simulink model "muv"  (Simulink 8.9)
settings: Solver=VariableStepAuto  StartTime=0.0  StopTime=10.0  RelTol=1e-3
settings Model: Creator=god  LastModifiedBy=muthu
settings DataIOCC: LimitDataPoints=off  SaveFormat=Dataset  SignalLoggingSaveFormat=Dataset
settings OptimizationCC: LifeSpan=auto
settings DebuggingCC: UnderspecifiedInitializationDetection=Simplified  MergeDetectMultiDrivingBlocksExec=error  FcnCallInpInsideContextMsg=error  StateNameClashWarn=none  SFUnexpectedBacktrackingDiag=error  SFNoUnconditionalDefaultTransitionDiag=error  SFExecutionAtInitializationDiag=warning
settings HardwareCC: ProdBitPerPointer=64  ProdBitPerSizeT=64  ProdBitPerPtrDiffT=64  ProdLargestAtomicFloat=Float  ProdIntDivRoundTo=Zero  ProdEndianess=LittleEndian  ProdWordSize=64  ProdHWDeviceType=Intel->x86-64 (Windows64)
settings ModelReferenceCC: PropagateSignalLabelsOutOfModel=on
settings GRTTargetCC: TargetLangStandard=C99 (ISO)  GeneratePreprocessorConditionals=Use local settings  CombineOutputUpdateFcns=on  GRTInterface=off
settings ConfigComp: CovMetricSettings=dwe  CovHtmlReporting=off  CovSaveCumulativeToWorkspaceVar=off  CovSaveSingleToWorkspaceVar=off  CovExternalEMLEnable=on

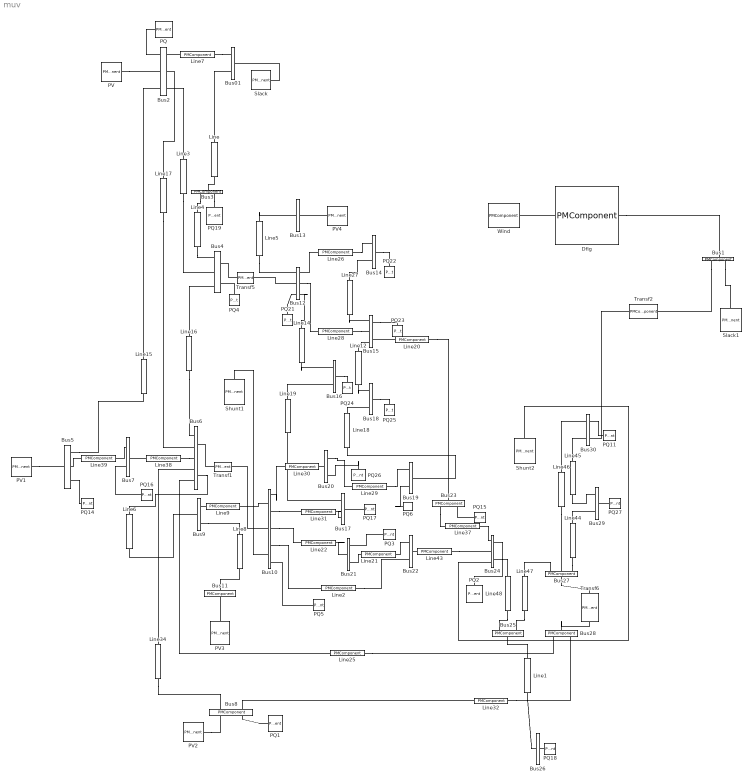
== system muv ==
  Bus01 : PMComponent  Tag=PSATblock  Description=Connection  PhysicalDomain=psatdomain  LeftPortType=p1  RightPortType=p1  LConnTagsString=__newl0  RConnTagsString=__newr0|__newr1  mask(Bus){in=1, out=2, p2q=132, p3_4q=[1.10  0.90], p5q=1, p6q=1}
      mask prompts: in "Number of inputs:"; out "Number of outputs:"; p2q "Voltage Rating [kV]"; p3_4q "Voltage initial guess [p.u.  rad]"; p5q "Area number"; p6q "Region number"
      mask help: Bus block.
      mask init:
      | fm_inout
      mask Callback p5q: fm_block
      mask Display: plot([0 1 1 0 0],[0 0 1 1 0])
  Bus1 : PMComponent  Tag=PSATblock  Description=Connection  PhysicalDomain=psatdomain  LeftPortType=p1  RightPortType=p1  LConnTagsString=__newl0|__newl1  RConnTagsString=__newr0  mask(Bus){in=2, out=1, p2q=33, p3_4q=[1.00  0.00], p5q=1, p6q=1}
      mask prompts: in "Number of inputs:"; out "Number of outputs:"; p2q "Voltage Rating [kV]"; p3_4q "Voltage initial guess [p.u.  rad]"; p5q "Area number"; p6q "Region number"
      mask help: Bus block.
      mask init:
      | fm_inout
      mask Callback p5q: fm_block
      mask Display: plot([0 1 1 0 0],[0 0 1 1 0])
  Bus10 : PMComponent  Tag=PSATblock  Description=Connection  PhysicalDomain=psatdomain  LeftPortType=p1  RightPortType=p1  LConnTagsString=__newl0|__newl1|__newl2  RConnTagsString=__newr0|__newr1|__newr2|__newr3|__newr4  mask(Bus){in=3, out=5, p2q=33, p3_4q=[1.00  0.00], p5q=1, p6q=1}
      mask prompts: in "Number of inputs:"; out "Number of outputs:"; p2q "Voltage Rating [kV]"; p3_4q "Voltage initial guess [p.u.  rad]"; p5q "Area number"; p6q "Region number"
      mask help: Bus block.
      mask init:
      | fm_inout
      mask Callback p5q: fm_block
      mask Display: plot([0 1 1 0 0],[0 0 1 1 0])
  Bus11 : PMComponent  Tag=PSATblock  Description=Connection  PhysicalDomain=psatdomain  LeftPortType=p1  RightPortType=p1  LConnTagsString=__newl0  RConnTagsString=__newr0  mask(Bus){in=1, out=1, p2q=132, p3_4q=[1.00  0.00], p5q=1, p6q=1}
      mask prompts: in "Number of inputs:"; out "Number of outputs:"; p2q "Voltage Rating [kV]"; p3_4q "Voltage initial guess [p.u.  rad]"; p5q "Area number"; p6q "Region number"
      mask help: Bus block.
      mask init:
      | fm_inout
      mask Callback p5q: fm_block
      mask Display: plot([0 1 1 0 0],[0 0 1 1 0])
  Bus12 : PMComponent  Tag=PSATblock  Description=Connection  PhysicalDomain=psatdomain  LeftPortType=p1  RightPortType=p1  LConnTagsString=__newl0|__newl1|__newl2  RConnTagsString=__newr0|__newr1|__newr2  mask(Bus){in=3, out=3, p2q=33, p3_4q=[1.00  0.00], p5q=1, p6q=1}
      mask prompts: in "Number of inputs:"; out "Number of outputs:"; p2q "Voltage Rating [kV]"; p3_4q "Voltage initial guess [p.u.  rad]"; p5q "Area number"; p6q "Region number"
      mask help: Bus block.
      mask init:
      | fm_inout
      mask Callback p5q: fm_block
      mask Display: plot([0 1 1 0 0],[0 0 1 1 0])
  Bus13 : PMComponent  Tag=PSATblock  Description=Connection  PhysicalDomain=psatdomain  LeftPortType=p1  RightPortType=p1  LConnTagsString=__newl0  RConnTagsString=__newr0  mask(Bus){in=1, out=1, p2q=11, p3_4q=[1.00  0.00], p5q=1, p6q=1}
      mask prompts: in "Number of inputs:"; out "Number of outputs:"; p2q "Voltage Rating [kV]"; p3_4q "Voltage initial guess [p.u.  rad]"; p5q "Area number"; p6q "Region number"
      mask help: Bus block.
      mask init:
      | fm_inout
      mask Callback p5q: fm_block
      mask Display: plot([0 1 1 0 0],[0 0 1 1 0])
  Bus14 : PMComponent  Tag=PSATblock  Description=Connection  PhysicalDomain=psatdomain  LeftPortType=p1  RightPortType=p1  LConnTagsString=__newl0|__newl1  RConnTagsString=__newr0  mask(Bus){in=2, out=1, p2q=33, p3_4q=[1.00  0.00], p5q=1, p6q=1}
      mask prompts: in "Number of inputs:"; out "Number of outputs:"; p2q "Voltage Rating [kV]"; p3_4q "Voltage initial guess [p.u.  rad]"; p5q "Area number"; p6q "Region number"
      mask help: Bus block.
      mask init:
      | fm_inout
      mask Callback p5q: fm_block
      mask Display: plot([0 1 1 0 0],[0 0 1 1 0])
  Bus15 : PMComponent  Tag=PSATblock  Description=Connection  PhysicalDomain=psatdomain  LeftPortType=p1  RightPortType=p1  LConnTagsString=__newl0|__newl1|__newl2  RConnTagsString=__newr0|__newr1  mask(Bus){in=3, out=2, p2q=33, p3_4q=[1.00  0.00], p5q=1, p6q=1}
      mask prompts: in "Number of inputs:"; out "Number of outputs:"; p2q "Voltage Rating [kV]"; p3_4q "Voltage initial guess [p.u.  rad]"; p5q "Area number"; p6q "Region number"
      mask help: Bus block.
      mask init:
      | fm_inout
      mask Callback p5q: fm_block
      mask Display: plot([0 1 1 0 0],[0 0 1 1 0])
  Bus16 : PMComponent  Tag=PSATblock  Description=Connection  PhysicalDomain=psatdomain  LeftPortType=p1  RightPortType=p1  LConnTagsString=__newl0|__newl1  RConnTagsString=__newr0  mask(Bus){in=2, out=1, p2q=33, p3_4q=[1.00  0.00], p5q=1, p6q=1}
      mask prompts: in "Number of inputs:"; out "Number of outputs:"; p2q "Voltage Rating [kV]"; p3_4q "Voltage initial guess [p.u.  rad]"; p5q "Area number"; p6q "Region number"
      mask help: Bus block.
      mask init:
      | fm_inout
      mask Callback p5q: fm_block
      mask Display: plot([0 1 1 0 0],[0 0 1 1 0])
  Bus17 : PMComponent  Tag=PSATblock  Description=Connection  PhysicalDomain=psatdomain  LeftPortType=p1  RightPortType=p1  LConnTagsString=__newl0|__newl1  RConnTagsString=__newr0  mask(Bus){in=2, out=1, p2q=33, p3_4q=[1.00  0.00], p5q=1, p6q=1}
      mask prompts: in "Number of inputs:"; out "Number of outputs:"; p2q "Voltage Rating [kV]"; p3_4q "Voltage initial guess [p.u.  rad]"; p5q "Area number"; p6q "Region number"
      mask help: Bus block.
      mask init:
      | fm_inout
      mask Callback p5q: fm_block
      mask Display: plot([0 1 1 0 0],[0 0 1 1 0])
  Bus18 : PMComponent  Tag=PSATblock  Description=Connection  PhysicalDomain=psatdomain  LeftPortType=p1  RightPortType=p1  LConnTagsString=__newl0|__newl1  RConnTagsString=__newr0  mask(Bus){in=2, out=1, p2q=33, p3_4q=[1.00  0.00], p5q=1, p6q=1}
      mask prompts: in "Number of inputs:"; out "Number of outputs:"; p2q "Voltage Rating [kV]"; p3_4q "Voltage initial guess [p.u.  rad]"; p5q "Area number"; p6q "Region number"
      mask help: Bus block.
      mask init:
      | fm_inout
      mask Callback p5q: fm_block
      mask Display: plot([0 1 1 0 0],[0 0 1 1 0])
  Bus19 : PMComponent  Tag=PSATblock  Description=Connection  PhysicalDomain=psatdomain  LeftPortType=p1  RightPortType=p1  LConnTagsString=__newl0|__newl1  RConnTagsString=__newr0  mask(Bus){in=2, out=1, p2q=33, p3_4q=[1.00  0.00], p5q=1, p6q=1}
      mask prompts: in "Number of inputs:"; out "Number of outputs:"; p2q "Voltage Rating [kV]"; p3_4q "Voltage initial guess [p.u.  rad]"; p5q "Area number"; p6q "Region number"
      mask help: Bus block.
      mask init:
      | fm_inout
      mask Callback p5q: fm_block
      mask Display: plot([0 1 1 0 0],[0 0 1 1 0])
  Bus2 : PMComponent  Tag=PSATblock  Description=Connection  PhysicalDomain=psatdomain  LeftPortType=p1  RightPortType=p1  LConnTagsString=__newl0|__newl1|__newl2  RConnTagsString=__newr0|__newr1|__newr2  mask(Bus){in=3, out=3, p2q=132, p3_4q=[1.00  0.00], p5q=1, p6q=1}
      mask prompts: in "Number of inputs:"; out "Number of outputs:"; p2q "Voltage Rating [kV]"; p3_4q "Voltage initial guess [p.u.  rad]"; p5q "Area number"; p6q "Region number"
      mask help: Bus block.
      mask init:
      | fm_inout
      mask Callback p5q: fm_block
      mask Display: plot([0 1 1 0 0],[0 0 1 1 0])
  Bus20 : PMComponent  Tag=PSATblock  Description=Connection  PhysicalDomain=psatdomain  LeftPortType=p1  RightPortType=p1  LConnTagsString=__newl0  RConnTagsString=__newr0|__newr1  mask(Bus){in=1, out=2, p2q=33, p3_4q=[1.00  0.00], p5q=1, p6q=1}
      mask prompts: in "Number of inputs:"; out "Number of outputs:"; p2q "Voltage Rating [kV]"; p3_4q "Voltage initial guess [p.u.  rad]"; p5q "Area number"; p6q "Region number"
      mask help: Bus block.
      mask init:
      | fm_inout
      mask Callback p5q: fm_block
      mask Display: plot([0 1 1 0 0],[0 0 1 1 0])
  Bus21 : PMComponent  Tag=PSATblock  Description=Connection  PhysicalDomain=psatdomain  LeftPortType=p1  RightPortType=p1  LConnTagsString=__newl0  RConnTagsString=__newr0|__newr1  mask(Bus){in=1, out=2, p2q=33, p3_4q=[1.00  0.00], p5q=1, p6q=1}
      mask prompts: in "Number of inputs:"; out "Number of outputs:"; p2q "Voltage Rating [kV]"; p3_4q "Voltage initial guess [p.u.  rad]"; p5q "Area number"; p6q "Region number"
      mask help: Bus block.
      mask init:
      | fm_inout
      mask Callback p5q: fm_block
      mask Display: plot([0 1 1 0 0],[0 0 1 1 0])
  Bus22 : PMComponent  Tag=PSATblock  Description=Connection  PhysicalDomain=psatdomain  LeftPortType=p1  RightPortType=p1  LConnTagsString=__newl0|__newl1  RConnTagsString=__newr0  mask(Bus){in=2, out=1, p2q=33, p3_4q=[1.00  0.00], p5q=1, p6q=1}
      mask prompts: in "Number of inputs:"; out "Number of outputs:"; p2q "Voltage Rating [kV]"; p3_4q "Voltage initial guess [p.u.  rad]"; p5q "Area number"; p6q "Region number"
      mask help: Bus block.
      mask init:
      | fm_inout
      mask Callback p5q: fm_block
      mask Display: plot([0 1 1 0 0],[0 0 1 1 0])
  Bus23 : PMComponent  Tag=PSATblock  Description=Connection  PhysicalDomain=psatdomain  LeftPortType=p1  RightPortType=p1  LConnTagsString=__newl0  RConnTagsString=__newr0|__newr1  mask(Bus){in=1, out=2, p2q=33, p3_4q=[1.00  0.00], p5q=1, p6q=1}
      mask prompts: in "Number of inputs:"; out "Number of outputs:"; p2q "Voltage Rating [kV]"; p3_4q "Voltage initial guess [p.u.  rad]"; p5q "Area number"; p6q "Region number"
      mask help: Bus block.
      mask init:
      | fm_inout
      mask Callback p5q: fm_block
      mask Display: plot([0 1 1 0 0],[0 0 1 1 0])
  Bus24 : PMComponent  Tag=PSATblock  Description=Connection  PhysicalDomain=psatdomain  LeftPortType=p1  RightPortType=p1  LConnTagsString=__newl0|__newl1|__newl2  RConnTagsString=__newr0|__newr1  mask(Bus){in=3, out=2, p2q=32, p3_4q=[1.00  0.00], p5q=1, p6q=1}
      mask prompts: in "Number of inputs:"; out "Number of outputs:"; p2q "Voltage Rating [kV]"; p3_4q "Voltage initial guess [p.u.  rad]"; p5q "Area number"; p6q "Region number"
      mask help: Bus block.
      mask init:
      | fm_inout
      mask Callback p5q: fm_block
      mask Display: plot([0 1 1 0 0],[0 0 1 1 0])
  Bus25 : PMComponent  Tag=PSATblock  Description=Connection  PhysicalDomain=psatdomain  LeftPortType=p1  RightPortType=p1  LConnTagsString=__newl0|__newl1  RConnTagsString=__newr0  mask(Bus){in=2, out=1, p2q=33, p3_4q=[1.00  0.00], p5q=1, p6q=1}
      mask prompts: in "Number of inputs:"; out "Number of outputs:"; p2q "Voltage Rating [kV]"; p3_4q "Voltage initial guess [p.u.  rad]"; p5q "Area number"; p6q "Region number"
      mask help: Bus block.
      mask init:
      | fm_inout
      mask Callback p5q: fm_block
      mask Display: plot([0 1 1 0 0],[0 0 1 1 0])
  Bus26 : PMComponent  Tag=PSATblock  Description=Connection  PhysicalDomain=psatdomain  LeftPortType=p1  RightPortType=p1  LConnTagsString=__newl0  RConnTagsString=__newr0  mask(Bus){in=1, out=1, p2q=33, p3_4q=[1.00  0.00], p5q=1, p6q=1}
      mask prompts: in "Number of inputs:"; out "Number of outputs:"; p2q "Voltage Rating [kV]"; p3_4q "Voltage initial guess [p.u.  rad]"; p5q "Area number"; p6q "Region number"
      mask help: Bus block.
      mask init:
      | fm_inout
      mask Callback p5q: fm_block
      mask Display: plot([0 1 1 0 0],[0 0 1 1 0])
  Bus27 : PMComponent  Tag=PSATblock  Description=Connection  PhysicalDomain=psatdomain  LeftPortType=p1  RightPortType=p1  LConnTagsString=__newl0  RConnTagsString=__newr0|__newr1|__newr2  mask(Bus){in=1, out=3, p2q=33, p3_4q=[1.00  0.00], p5q=1, p6q=1}
      mask prompts: in "Number of inputs:"; out "Number of outputs:"; p2q "Voltage Rating [kV]"; p3_4q "Voltage initial guess [p.u.  rad]"; p5q "Area number"; p6q "Region number"
      mask help: Bus block.
      mask init:
      | fm_inout
      mask Callback p5q: fm_block
      mask Display: plot([0 1 1 0 0],[0 0 1 1 0])
  Bus28 : PMComponent  Tag=PSATblock  Description=Connection  PhysicalDomain=psatdomain  LeftPortType=p1  RightPortType=p1  LConnTagsString=__newl0|__newl1  RConnTagsString=__newr0  mask(Bus){in=2, out=1, p2q=132, p3_4q=[1.00  0.00], p5q=1, p6q=1}
      mask prompts: in "Number of inputs:"; out "Number of outputs:"; p2q "Voltage Rating [kV]"; p3_4q "Voltage initial guess [p.u.  rad]"; p5q "Area number"; p6q "Region number"
      mask help: Bus block.
      mask init:
      | fm_inout
      mask Callback p5q: fm_block
      mask Display: plot([0 1 1 0 0],[0 0 1 1 0])
  Bus29 : PMComponent  Tag=PSATblock  Description=Connection  PhysicalDomain=psatdomain  LeftPortType=p1  RightPortType=p1  LConnTagsString=__newl0|__newl1  RConnTagsString=__newr0  mask(Bus){in=2, out=1, p2q=33, p3_4q=[1.00  0.00], p5q=1, p6q=1}
      mask prompts: in "Number of inputs:"; out "Number of outputs:"; p2q "Voltage Rating [kV]"; p3_4q "Voltage initial guess [p.u.  rad]"; p5q "Area number"; p6q "Region number"
      mask help: Bus block.
      mask init:
      | fm_inout
      mask Callback p5q: fm_block
      mask Display: plot([0 1 1 0 0],[0 0 1 1 0])
  Bus3 : PMComponent  Tag=PSATblock  Description=Connection  PhysicalDomain=psatdomain  LeftPortType=p1  RightPortType=p1  LConnTagsString=__newl0  RConnTagsString=__newr0|__newr1  mask(Bus){in=1, out=2, p2q=132, p3_4q=[1.00  0.00], p5q=1, p6q=1}
      mask prompts: in "Number of inputs:"; out "Number of outputs:"; p2q "Voltage Rating [kV]"; p3_4q "Voltage initial guess [p.u.  rad]"; p5q "Area number"; p6q "Region number"
      mask help: Bus block.
      mask init:
      | fm_inout
      mask Callback p5q: fm_block
      mask Display: plot([0 1 1 0 0],[0 0 1 1 0])
  Bus30 : PMComponent  Tag=PSATblock  Description=Connection  PhysicalDomain=psatdomain  LeftPortType=p1  RightPortType=p1  LConnTagsString=__newl0|__newl1  RConnTagsString=__newr0|__newr1  mask(Bus){in=2, out=2, p2q=33, p3_4q=[1.00  0.00], p5q=1, p6q=1}
      mask prompts: in "Number of inputs:"; out "Number of outputs:"; p2q "Voltage Rating [kV]"; p3_4q "Voltage initial guess [p.u.  rad]"; p5q "Area number"; p6q "Region number"
      mask help: Bus block.
      mask init:
      | fm_inout
      mask Callback p5q: fm_block
      mask Display: plot([0 1 1 0 0],[0 0 1 1 0])
  Bus4 : PMComponent  Tag=PSATblock  Description=Connection  PhysicalDomain=psatdomain  LeftPortType=p1  RightPortType=p1  LConnTagsString=__newl0|__newl1|__newl2  RConnTagsString=__newr0|__newr1  mask(Bus){in=3, out=2, p2q=132, p3_4q=[1   0.00], p5q=1, p6q=1}
      mask prompts: in "Number of inputs:"; out "Number of outputs:"; p2q "Voltage Rating [kV]"; p3_4q "Voltage initial guess [p.u.   rad]"; p5q "Area number"; p6q "Region number"
      mask help: Bus block
      mask init:
      | fm_inout
      mask Callback p5q: fm_block
      mask Display: plot([0 1 1 0 0],[0 0 1 1 0])
  Bus5 : PMComponent  Tag=PSATblock  Description=Connection  PhysicalDomain=psatdomain  LeftPortType=p1  RightPortType=p1  LConnTagsString=__newl0  RConnTagsString=__newr0|__newr1|__newr2  mask(Bus){in=1, out=3, p2q=132, p3_4q=[1.00   0.00], p5q=1, p6q=1}
      mask prompts: in "Number of inputs:"; out "Number of outputs:"; p2q "Voltage Rating [kV]"; p3_4q "Voltage initial guess [p.u.   rad]"; p5q "Area number"; p6q "Region number"
      mask help: Bus block
      mask init:
      | fm_inout
      mask Callback p5q: fm_block
      mask Display: plot([0 1 1 0 0],[0 0 1 1 0])
  Bus6 : PMComponent  Tag=PSATblock  Description=Connection  PhysicalDomain=psatdomain  LeftPortType=p1  RightPortType=p1  LConnTagsString=__newl0|__newl1|__newl2|__newl3|__newl4  RConnTagsString=__newr0|__newr1  mask(Bus){in=5, out=2, p2q=132, p3_4q=[1.00   0.00], p5q=1, p6q=1}
      mask prompts: in "Number of inputs:"; out "Number of outputs:"; p2q "Voltage Rating [kV]"; p3_4q "Voltage initial guess [p.u.   rad]"; p5q "Area number"; p6q "Region number"
      mask help: Bus block
      mask init:
      | fm_inout
      mask Callback p5q: fm_block
      mask Display: plot([0 1 1 0 0],[0 0 1 1 0])
  Bus7 : PMComponent  Tag=PSATblock  Description=Connection  PhysicalDomain=psatdomain  LeftPortType=p1  RightPortType=p1  LConnTagsString=__newl0|__newl1  RConnTagsString=__newr0  mask(Bus){in=2, out=1, p2q=132, p3_4q=[1.00   0.00], p5q=1, p6q=1}
      mask prompts: in "Number of inputs:"; out "Number of outputs:"; p2q "Voltage Rating [kV]"; p3_4q "Voltage initial guess [p.u.   rad]"; p5q "Area number"; p6q "Region number"
      mask help: Bus block
      mask init:
      | fm_inout
      mask Callback p5q: fm_block
      mask Display: plot([0 1 1 0 0],[0 0 1 1 0])
  Bus8 : PMComponent  Tag=PSATblock  Description=Connection  PhysicalDomain=psatdomain  LeftPortType=p1  RightPortType=p1  LConnTagsString=__newl0|__newl1  RConnTagsString=__newr0|__newr1  mask(Bus){in=2, out=2, p2q=132, p3_4q=[1.00   0.00], p5q=1, p6q=1}
      mask prompts: in "Number of inputs:"; out "Number of outputs:"; p2q "Voltage Rating [kV]"; p3_4q "Voltage initial guess [p.u.   rad]"; p5q "Area number"; p6q "Region number"
      mask help: Bus block
      mask init:
      | fm_inout
      mask Callback p5q: fm_block
      mask Display: plot([0 1 1 0 0],[0 0 1 1 0])
  Bus9 : PMComponent  Tag=PSATblock  Description=Connection  PhysicalDomain=psatdomain  LeftPortType=p1  RightPortType=p1  LConnTagsString=__newl0  RConnTagsString=__newr0|__newr1  mask(Bus){in=1, out=2, p2q=1, p3_4q=[1.00  0.00], p5q=1, p6q=1}
      mask prompts: in "Number of inputs:"; out "Number of outputs:"; p2q "Voltage Rating [kV]"; p3_4q "Voltage initial guess [p.u.  rad]"; p5q "Area number"; p6q "Region number"
      mask help: Bus block.
      mask init:
      | fm_inout
      mask Callback p5q: fm_block
      mask Display: plot([0 1 1 0 0],[0 0 1 1 0])
  Dfig : PMComponent  Tag=PSATblock  Description=Wind Turbines  PhysicalDomain=psatdomain  LeftPortType=p1  RightPortType=p1  LConnTagsString=__newl0  RConnTagsString=__newr0  mask(Dfig){p3_4_5q=[100   33   50], p6_7q=[0.01  0.10], p8_9q=[0.01  0.08], p10q=3.00, p11q=3, p12_13q=[10 3], p14q=10, p15q=0.01, p17_19q=[4 1/89], p16_18q=[75.00  3], p20_21q=[1.00  0.00], p22_23q=[0.7  -0.7], p24q=1, p25q=on}
      mask prompts: p3_4_5q "Power, Voltage and Frequency Ratings [MVA, kV, Hz]"; p6_7q "Stator Resistance Rs and Reactance Xs [p.u.  p.u.]"; p8_9q "Rotor Resitance Rr and Reactance Xr [p.u. p.u.]"; p10q "Magnetization Reactance Xm [p.u.]"; p11q "Inertia Constants Hm  [kWs/kVA]"; p12_13q "Pitch control gain and time constant  Kp, Tp [p.u.  s]"; p14q "Voltage control gain Kv [p.u.]"; p15q "Power Control time constant Te [s]"; p17_19q "Number of poles p and gear box ratio [int  -]"; p16_18q "Blade length and number [m int]"; p20_21q "Pmax and Pmin [p.u.  p.u.]"; p22_23q "Qmax and Qmin [p.u.  p.u.]"; p24q "Number of wind generators that compose the park"; p25q "Connected"
      mask help: This block defines a variable speed wind turbine with doubly fed induction generator.
      mask init:
      | [x,y] = fm_draw('circle');
      | [xh,yh] = fm_draw('helix');
      mask Callback p25q: fm_block
      mask Display:
      | plot(1.4*x,1.4*y,[0,-2],[0 0],[-2 -3 -3 -2 -2],[-1 -1 1 1 -1],[-3 -5],[0 0],[1.4 3.5],[0 0],1,4.35,[0 0 1.075],[-1 -3.25 -3.25],[2.05  2.05],[0 -2.15])
      | plot(1.5*[0.3 0.3]+2.5,0.5*[-1.7 2.7]-3.5,1.5*[ -0.95  -0.95]+2.5,0.5*[-1.7 2.7]-3.5,1.5*[0 0.2]+2.5,0.5*[0.5 0.5]-3.5)
      | plot(1.5*[0.3 -0.95]+2.5,0.5*[2.7 2.7]-3.5,1.5*[0.3 -0.95]+2.5,0.5*[-1.7 -1.7]-3.5)
      | color('blue')
      | plot(x,y)
      | color('cyan')
      | plot(xh-4,3*yh)
      | color('magenta')
      | plot(1.5*[0 0]+2.5,0.5*[-0.5 1.5]-3.5,1.5*[0 -0.2]+2.5,0.5*[-0.5 -0.5]-3.5,1.5*[0 -0.65]+2.5,0.5*[1.5 1.5]-3.5)
      | plot(1.5*[-0.2 -0.2]+2.5,0.5*[-1 0]-3.5,1.5*[-0.2 -0.45]+2.5,0.5*[-1 -0.5]-3.5,1.5*[-0.2 -0.45]+2.5,0.5*[0 -0.5]-3.5,1.5*[-0.45 -0.45]+2.5,0.5*[-1 0]-3.5)
      | plot(1.5*[-0.2 -0.2]+2.5,0.5*[2 1]-3.5,1.5*[-0.45 -0.45]+2.5,0.5*[2 1]-3.5,1.5*[-0.45 -0.2]+2.5,0.5*[2 1.5]-3.5,1.5*[-0.45 -0.2]+2.5,0.5*[1 1.5]-3.5)
      | plot(1.5*[-0.65 -0.65]+2.5,0.5*[-0.5 1.5]-3.5,1.5*[-0.45 -0.65]+2.5,0.5*[-0.5 -0.5]-3.5,1.5*[-0.45 -0.65]+2.5,0.5*[1.5 1.5]-3.5)
      | plot(1.5*[-0.65 -0.85]+2.5,0.5*[0.5 0.5]-3.5,1.5*[-0.3 -0.3]+2.5,0.5*[1.7 2.2]-3.5,1.5*[-0.325 -0.275]+2.5,0.5*[1.975 1.975]-3.5)
  Line : PMComponent  Tag=PSATblock  Description=Power Flow  PhysicalDomain=psatdomain  LeftPortType=p1  RightPortType=p1  LConnTagsString=__newl0  RConnTagsString=__newr0  mask(Line){p3_4_5q=[130  132 50], p6q=0, p8q=0.0452, p9q=0.1852, p10q=0.04080, p13_14_15q=[0.0  0.0  0.0], p16q=on}
      mask prompts: p3_4_5q "Power, Voltage and Frequency Ratings [MVA, kV, Hz]"; p6q "Length of line [km] (0 for p.u. parameters)"; p8q "Resistance [p.u. (Ohms/km)]"; p9q "Reactance [p.u. (H/km)]"; p10q "Susceptance [p.u. (F/km)]"; p13_14_15q "Imax, Pmax and Smax [p.u., p.u., p.u.]"; p16q "Connected"
      mask help: This block defines a pi model for a tree phase line.
      mask init:
      | [xp,yp] = fm_draw('pi');
      mask Callback p16q: fm_block
      mask Display:
      | plot([-1  1  1 -1 -1],[-0.2 -0.2 0.2 0.2 -0.2])
      | color('blue')
      | plot(0.35*xp,0.2*yp)
  Line1 : PMComponent  Tag=PSATblock  Description=Power Flow  PhysicalDomain=psatdomain  LeftPortType=p1  RightPortType=p1  LConnTagsString=__newl0  RConnTagsString=__newr0  mask(Line){p3_4_5q=[16 33 50], p6q=0, p8q=0.05, p9q=0.10, p10q=0, p13_14_15q=[0.0  0.0  0.0], p16q=on}
      mask prompts: p3_4_5q "Power, Voltage and Frequency Ratings [MVA, kV, Hz]"; p6q "Length of line [km] (0 for p.u. parameters)"; p8q "Resistance [p.u. (Ohms/km)]"; p9q "Reactance [p.u. (H/km)]"; p10q "Susceptance [p.u. (F/km)]"; p13_14_15q "Imax, Pmax and Smax [p.u., p.u., p.u.]"; p16q "Connected"
      mask help: This block defines a pi model for a tree phase line.
      mask init:
      | [xp,yp] = fm_draw('pi');
      mask Callback p16q: fm_block
      mask Display:
      | plot([-1  1  1 -1 -1],[-0.2 -0.2 0.2 0.2 -0.2])
      | color('blue')
      | plot(0.35*xp,0.2*yp)
  Line12 : PMComponent  Tag=PSATblock  Description=Power Flow  PhysicalDomain=psatdomain  LeftPortType=p1  RightPortType=p1  LConnTagsString=__newl0  RConnTagsString=__newr0  mask(Line){p3_4_5q=[16 33  50], p6q=0, p8q=0.1073, p9q=0.2185, p10q=0, p13_14_15q=[0.0  0.0  0.0], p16q=on}
      mask prompts: p3_4_5q "Power, Voltage and Frequency Ratings [MVA, kV, Hz]"; p6q "Length of line [km] (0 for p.u. parameters)"; p8q "Resistance [p.u. (Ohms/km)]"; p9q "Reactance [p.u. (H/km)]"; p10q "Susceptance [p.u. (F/km)]"; p13_14_15q "Imax, Pmax and Smax [p.u., p.u., p.u.]"; p16q "Connected"
      mask help: This block defines a pi model for a tree phase line.
      mask init:
      | [xp,yp] = fm_draw('pi');
      mask Callback p16q: fm_block
      mask Display:
      | plot([-1  1  1 -1 -1],[-0.2 -0.2 0.2 0.2 -0.2])
      | color('blue')
      | plot(0.35*xp,0.2*yp)
  Line14 : PMComponent  Tag=PSATblock  Description=Power Flow  PhysicalDomain=psatdomain  LeftPortType=p1  RightPortType=p1  LConnTagsString=__newl0  RConnTagsString=__newr0  mask(Line){p3_4_5q=[32  33  50], p6q=0, p8q=0.0945, p9q=0.1987, p10q=0, p13_14_15q=[0.0  0.0  0.0], p16q=on}
      mask prompts: p3_4_5q "Power, Voltage and Frequency Ratings [MVA, kV, Hz]"; p6q "Length of line [km] (0 for p.u. parameters)"; p8q "Resistance [p.u. (Ohms/km)]"; p9q "Reactance [p.u. (H/km)]"; p10q "Susceptance [p.u. (F/km)]"; p13_14_15q "Imax, Pmax and Smax [p.u., p.u., p.u.]"; p16q "Connected"
      mask help: This block defines a pi model for a tree phase line.
      mask init:
      | [xp,yp] = fm_draw('pi');
      mask Callback p16q: fm_block
      mask Display:
      | plot([-1  1  1 -1 -1],[-0.2 -0.2 0.2 0.2 -0.2])
      | color('blue')
      | plot(0.35*xp,0.2*yp)
  Line15 : PMComponent  Tag=PSATblock  Description=Power Flow  PhysicalDomain=psatdomain  LeftPortType=p1  RightPortType=p1  LConnTagsString=__newl0  RConnTagsString=__newr0  mask(Line){p3_4_5q=[130 132 50], p6q=0, p8q=0.0472, p9q=0.1983, p10q=0.0418, p13_14_15q=[0.0  0.0  0.0], p16q=on}
      mask prompts: p3_4_5q "Power, Voltage and Frequency Ratings [MVA, kV, Hz]"; p6q "Length of line [km] (0 for p.u. parameters)"; p8q "Resistance [p.u. (Ohms/km)]"; p9q "Reactance [p.u. (H/km)]"; p10q "Susceptance [p.u. (F/km)]"; p13_14_15q "Imax, Pmax and Smax [p.u., p.u., p.u.]"; p16q "Connected"
      mask help: This block defines a pi model for a tree phase line.
      mask init:
      | [xp,yp] = fm_draw('pi');
      mask Callback p16q: fm_block
      mask Display:
      | plot([-1  1  1 -1 -1],[-0.2 -0.2 0.2 0.2 -0.2])
      | color('blue')
      | plot(0.35*xp,0.2*yp)
  Line16 : PMComponent  Tag=PSATblock  Description=Power Flow  PhysicalDomain=psatdomain  LeftPortType=p1  RightPortType=p1  LConnTagsString=__newl0  RConnTagsString=__newr0  mask(Line){p3_4_5q=[90  132  50], p6q=0, p8q=0.0119, p9q=0.0414, p10q=0.0045, p13_14_15q=[0.0  0.0  0.0], p16q=on}
      mask prompts: p3_4_5q "Power, Voltage and Frequency Ratings [MVA, kV, Hz]"; p6q "Length of line [km] (0 for p.u. parameters)"; p8q "Resistance [p.u. (Ohms/km)]"; p9q "Reactance [p.u. (H/km)]"; p10q "Susceptance [p.u. (F/km)]"; p13_14_15q "Imax, Pmax and Smax [p.u., p.u., p.u.]"; p16q "Connected"
      mask help: This block defines a pi model for a tree phase line.
      mask init:
      | [xp,yp] = fm_draw('pi');
      mask Callback p16q: fm_block
      mask Display:
      | plot([-1  1  1 -1 -1],[-0.2 -0.2 0.2 0.2 -0.2])
      | color('blue')
      | plot(0.35*xp,0.2*yp)
  Line17 : PMComponent  Tag=PSATblock  Description=Power Flow  PhysicalDomain=psatdomain  LeftPortType=p1  RightPortType=p1  LConnTagsString=__newl0  RConnTagsString=__newr0  mask(Line){p3_4_5q=[65  132  50], p6q=0, p8q=0.0581, p9q=0.1763, p10q=0.0374, p13_14_15q=[0.0  0.0  0.0], p16q=on}
      mask prompts: p3_4_5q "Power, Voltage and Frequency Ratings [MVA, kV, Hz]"; p6q "Length of line [km] (0 for p.u. parameters)"; p8q "Resistance [p.u. (Ohms/km)]"; p9q "Reactance [p.u. (H/km)]"; p10q "Susceptance [p.u. (F/km)]"; p13_14_15q "Imax, Pmax and Smax [p.u., p.u., p.u.]"; p16q "Connected"
      mask help: This block defines a pi model for a tree phase line.
      mask init:
      | [xp,yp] = fm_draw('pi');
      mask Callback p16q: fm_block
      mask Display:
      | plot([-1  1  1 -1 -1],[-0.2 -0.2 0.2 0.2 -0.2])
      | color('blue')
      | plot(0.35*xp,0.2*yp)
  Line18 : PMComponent  Tag=PSATblock  Description=Power Flow  PhysicalDomain=psatdomain  LeftPortType=p1  RightPortType=p1  LConnTagsString=__newl0  RConnTagsString=__newr0  mask(Line){p3_4_5q=[16 33  50], p6q=0, p8q=0.0639, p9q=0.1292, p10q=0, p13_14_15q=[0.0  0.0  0.0], p16q=on}
      mask prompts: p3_4_5q "Power, Voltage and Frequency Ratings [MVA, kV, Hz]"; p6q "Length of line [km] (0 for p.u. parameters)"; p8q "Resistance [p.u. (Ohms/km)]"; p9q "Reactance [p.u. (H/km)]"; p10q "Susceptance [p.u. (F/km)]"; p13_14_15q "Imax, Pmax and Smax [p.u., p.u., p.u.]"; p16q "Connected"
      mask help: This block defines a pi model for a tree phase line.
      mask init:
      | [xp,yp] = fm_draw('pi');
      mask Callback p16q: fm_block
      mask Display:
      | plot([-1  1  1 -1 -1],[-0.2 -0.2 0.2 0.2 -0.2])
      | color('blue')
      | plot(0.35*xp,0.2*yp)
  Line19 : PMComponent  Tag=PSATblock  Description=Power Flow  PhysicalDomain=psatdomain  LeftPortType=p1  RightPortType=p1  LConnTagsString=__newl0  RConnTagsString=__newr0  mask(Line){p3_4_5q=[16  33  50], p6q=0, p8q=0.0824, p9q=0.1932, p10q=0, p13_14_15q=[0.0  0.0  0.0], p16q=on}
      mask prompts: p3_4_5q "Power, Voltage and Frequency Ratings [MVA, kV, Hz]"; p6q "Length of line [km] (0 for p.u. parameters)"; p8q "Resistance [p.u. (Ohms/km)]"; p9q "Reactance [p.u. (H/km)]"; p10q "Susceptance [p.u. (F/km)]"; p13_14_15q "Imax, Pmax and Smax [p.u., p.u., p.u.]"; p16q "Connected"
      mask help: This block defines a pi model for a tree phase line.
      mask init:
      | [xp,yp] = fm_draw('pi');
      mask Callback p16q: fm_block
      mask Display:
      | plot([-1  1  1 -1 -1],[-0.2 -0.2 0.2 0.2 -0.2])
      | color('blue')
      | plot(0.35*xp,0.2*yp)
  Line2 : PMComponent  Tag=PSATblock  Description=Power Flow  PhysicalDomain=psatdomain  LeftPortType=p1  RightPortType=p1  LConnTagsString=__newl0  RConnTagsString=__newr0  mask(Line){p3_4_5q=[32 33  50], p6q=0, p8q=0.0727, p9q=0.1499, p10q=0, p13_14_15q=[0.0  0.0  0.0], p16q=on}
      mask prompts: p3_4_5q "Power, Voltage and Frequency Ratings [MVA, kV, Hz]"; p6q "Length of line [km] (0 for p.u. parameters)"; p8q "Resistance [p.u. (Ohms/km)]"; p9q "Reactance [p.u. (H/km)]"; p10q "Susceptance [p.u. (F/km)]"; p13_14_15q "Imax, Pmax and Smax [p.u., p.u., p.u.]"; p16q "Connected"
      mask help: This block defines a pi model for a tree phase line.
      mask init:
      | [xp,yp] = fm_draw('pi');
      mask Callback p16q: fm_block
      mask Display:
      | plot([-1  1  1 -1 -1],[-0.2 -0.2 0.2 0.2 -0.2])
      | color('blue')
      | plot(0.35*xp,0.2*yp)
  Line20 : PMComponent  Tag=PSATblock  Description=Power Flow  PhysicalDomain=psatdomain  LeftPortType=p1  RightPortType=p1  LConnTagsString=__newl0  RConnTagsString=__newr0  mask(Line){p3_4_5q=[16  33  50], p6q=0, p8q=0, p9q=0.202, p10q=0, p13_14_15q=[0.0  0.0  0.0], p16q=on}
      mask prompts: p3_4_5q "Power, Voltage and Frequency Ratings [MVA, kV, Hz]"; p6q "Length of line [km] (0 for p.u. parameters)"; p8q "Resistance [p.u. (Ohms/km)]"; p9q "Reactance [p.u. (H/km)]"; p10q "Susceptance [p.u. (F/km)]"; p13_14_15q "Imax, Pmax and Smax [p.u., p.u., p.u.]"; p16q "Connected"
      mask help: This block defines a pi model for a tree phase line.
      mask init:
      | [xp,yp] = fm_draw('pi');
      mask Callback p16q: fm_block
      mask Display:
      | plot([-1  1  1 -1 -1],[-0.2 -0.2 0.2 0.2 -0.2])
      | color('blue')
      | plot(0.35*xp,0.2*yp)
  Line21 : PMComponent  Tag=PSATblock  Description=Power Flow  PhysicalDomain=psatdomain  LeftPortType=p1  RightPortType=p1  LConnTagsString=__newl0  RConnTagsString=__newr0  mask(Line){p3_4_5q=[32 33  50], p6q=0, p8q=0.0116, p9q=0.0236, p10q=0, p13_14_15q=[0.0  0.0  0.0], p16q=on}
      mask prompts: p3_4_5q "Power, Voltage and Frequency Ratings [MVA, kV, Hz]"; p6q "Length of line [km] (0 for p.u. parameters)"; p8q "Resistance [p.u. (Ohms/km)]"; p9q "Reactance [p.u. (H/km)]"; p10q "Susceptance [p.u. (F/km)]"; p13_14_15q "Imax, Pmax and Smax [p.u., p.u., p.u.]"; p16q "Connected"
      mask help: This block defines a pi model for a tree phase line.
      mask init:
      | [xp,yp] = fm_draw('pi');
      mask Callback p16q: fm_block
      mask Display:
      | plot([-1  1  1 -1 -1],[-0.2 -0.2 0.2 0.2 -0.2])
      | color('blue')
      | plot(0.35*xp,0.2*yp)
  Line22 : PMComponent  Tag=PSATblock  Description=Power Flow  PhysicalDomain=psatdomain  LeftPortType=p1  RightPortType=p1  LConnTagsString=__newl0  RConnTagsString=__newr0  mask(Line){p3_4_5q=[32  33  50], p6q=0, p8q=0.0348, p9q=0.0749, p10q=0, p13_14_15q=[0.0  0.0  0.0], p16q=on}
      mask prompts: p3_4_5q "Power, Voltage and Frequency Ratings [MVA, kV, Hz]"; p6q "Length of line [km] (0 for p.u. parameters)"; p8q "Resistance [p.u. (Ohms/km)]"; p9q "Reactance [p.u. (H/km)]"; p10q "Susceptance [p.u. (F/km)]"; p13_14_15q "Imax, Pmax and Smax [p.u., p.u., p.u.]"; p16q "Connected"
      mask help: This block defines a pi model for a tree phase line.
      mask init:
      | [xp,yp] = fm_draw('pi');
      mask Callback p16q: fm_block
      mask Display:
      | plot([-1  1  1 -1 -1],[-0.2 -0.2 0.2 0.2 -0.2])
      | color('blue')
      | plot(0.35*xp,0.2*yp)
  Line25 : PMComponent  Tag=PSATblock  Description=Power Flow  PhysicalDomain=psatdomain  LeftPortType=p1  RightPortType=p1  LConnTagsString=__newl0  RConnTagsString=__newr0  mask(Line){p3_4_5q=[32 132 50], p6q=0, p8q=0.0169, p9q=0.0599, p10q=0.013, p13_14_15q=[0.0  0.0  0.0], p16q=on}
      mask prompts: p3_4_5q "Power, Voltage and Frequency Ratings [MVA, kV, Hz]"; p6q "Length of line [km] (0 for p.u. parameters)"; p8q "Resistance [p.u. (Ohms/km)]"; p9q "Reactance [p.u. (H/km)]"; p10q "Susceptance [p.u. (F/km)]"; p13_14_15q "Imax, Pmax and Smax [p.u., p.u., p.u.]"; p16q "Connected"
      mask help: This block defines a pi model for a tree phase line.
      mask init:
      | [xp,yp] = fm_draw('pi');
      mask Callback p16q: fm_block
      mask Display:
      | plot([-1  1  1 -1 -1],[-0.2 -0.2 0.2 0.2 -0.2])
      | color('blue')
      | plot(0.35*xp,0.2*yp)
  Line26 : PMComponent  Tag=PSATblock  Description=Power Flow  PhysicalDomain=psatdomain  LeftPortType=p1  RightPortType=p1  LConnTagsString=__newl0  RConnTagsString=__newr0  mask(Line){p3_4_5q=[32  33 50], p6q=0, p8q=0.1231, p9q=0.2559, p10q=0, p13_14_15q=[0.0  0.0  0.0], p16q=on}
      mask prompts: p3_4_5q "Power, Voltage and Frequency Ratings [MVA, kV, Hz]"; p6q "Length of line [km] (0 for p.u. parameters)"; p8q "Resistance [p.u. (Ohms/km)]"; p9q "Reactance [p.u. (H/km)]"; p10q "Susceptance [p.u. (F/km)]"; p13_14_15q "Imax, Pmax and Smax [p.u., p.u., p.u.]"; p16q "Connected"
      mask help: This block defines a pi model for a tree phase line.
      mask init:
      | [xp,yp] = fm_draw('pi');
      mask Callback p16q: fm_block
      mask Display:
      | plot([-1  1  1 -1 -1],[-0.2 -0.2 0.2 0.2 -0.2])
      | color('blue')
      | plot(0.35*xp,0.2*yp)
  Line27 : PMComponent  Tag=PSATblock  Description=Power Flow  PhysicalDomain=psatdomain  LeftPortType=p1  RightPortType=p1  LConnTagsString=__newl0  RConnTagsString=__newr0  mask(Line){p3_4_5q=[16  33  50], p6q=0, p8q=0.221, p9q=0.1997, p10q=0, p13_14_15q=[0.0  0.0  0.0], p16q=on}
      mask prompts: p3_4_5q "Power, Voltage and Frequency Ratings [MVA, kV, Hz]"; p6q "Length of line [km] (0 for p.u. parameters)"; p8q "Resistance [p.u. (Ohms/km)]"; p9q "Reactance [p.u. (H/km)]"; p10q "Susceptance [p.u. (F/km)]"; p13_14_15q "Imax, Pmax and Smax [p.u., p.u., p.u.]"; p16q "Connected"
      mask help: This block defines a pi model for a tree phase line.
      mask init:
      | [xp,yp] = fm_draw('pi');
      mask Callback p16q: fm_block
      mask Display:
      | plot([-1  1  1 -1 -1],[-0.2 -0.2 0.2 0.2 -0.2])
      | color('blue')
      | plot(0.35*xp,0.2*yp)
  Line28 : PMComponent  Tag=PSATblock  Description=Power Flow  PhysicalDomain=psatdomain  LeftPortType=p1  RightPortType=p1  LConnTagsString=__newl0  RConnTagsString=__newr0  mask(Line){p3_4_5q=[32  33  50], p6q=0, p8q=0.0662, p9q=0.1304, p10q=0, p13_14_15q=[0.0  0.0  0.0], p16q=on}
      mask prompts: p3_4_5q "Power, Voltage and Frequency Ratings [MVA, kV, Hz]"; p6q "Length of line [km] (0 for p.u. parameters)"; p8q "Resistance [p.u. (Ohms/km)]"; p9q "Reactance [p.u. (H/km)]"; p10q "Susceptance [p.u. (F/km)]"; p13_14_15q "Imax, Pmax and Smax [p.u., p.u., p.u.]"; p16q "Connected"
      mask help: This block defines a pi model for a tree phase line.
      mask init:
      | [xp,yp] = fm_draw('pi');
      mask Callback p16q: fm_block
      mask Display:
      | plot([-1  1  1 -1 -1],[-0.2 -0.2 0.2 0.2 -0.2])
      | color('blue')
      | plot(0.35*xp,0.2*yp)
  Line29 : PMComponent  Tag=PSATblock  Description=Power Flow  PhysicalDomain=psatdomain  LeftPortType=p1  RightPortType=p1  LConnTagsString=__newl0  RConnTagsString=__newr0  mask(Line){p3_4_5q=[32  33  50], p6q=0, p8q=0.034, p9q=0.068, p10q=0, p13_14_15q=[0.0  0.0  0.0], p16q=on}
      mask prompts: p3_4_5q "Power, Voltage and Frequency Ratings [MVA, kV, Hz]"; p6q "Length of line [km] (0 for p.u. parameters)"; p8q "Resistance [p.u. (Ohms/km)]"; p9q "Reactance [p.u. (H/km)]"; p10q "Susceptance [p.u. (F/km)]"; p13_14_15q "Imax, Pmax and Smax [p.u., p.u., p.u.]"; p16q "Connected"
      mask help: This block defines a pi model for a tree phase line.
      mask init:
      | [xp,yp] = fm_draw('pi');
      mask Callback p16q: fm_block
      mask Display:
      | plot([-1  1  1 -1 -1],[-0.2 -0.2 0.2 0.2 -0.2])
      | color('blue')
      | plot(0.35*xp,0.2*yp)
  Line3 : PMComponent  Tag=PSATblock  Description=Power Flow  PhysicalDomain=psatdomain  LeftPortType=p1  RightPortType=p1  LConnTagsString=__newl0  RConnTagsString=__newr0  mask(Line){p3_4_5q=[65  130  50], p6q=0, p8q=0.057, p9q=0.1737, p10q=0.0368, p13_14_15q=[0.0  0.0  0.0], p16q=on}
      mask prompts: p3_4_5q "Power, Voltage and Frequency Ratings [MVA, kV, Hz]"; p6q "Length of line [km] (0 for p.u. parameters)"; p8q "Resistance [p.u. (Ohms/km)]"; p9q "Reactance [p.u. (H/km)]"; p10q "Susceptance [p.u. (F/km)]"; p13_14_15q "Imax, Pmax and Smax [p.u., p.u., p.u.]"; p16q "Connected"
      mask help: This block defines a pi model for a tree phase line.
      mask init:
      | [xp,yp] = fm_draw('pi');
      mask Callback p16q: fm_block
      mask Display:
      | plot([-1  1  1 -1 -1],[-0.2 -0.2 0.2 0.2 -0.2])
      | color('blue')
      | plot(0.35*xp,0.2*yp)
  Line30 : PMComponent  Tag=PSATblock  Description=Power Flow  PhysicalDomain=psatdomain  LeftPortType=p1  RightPortType=p1  LConnTagsString=__newl0  RConnTagsString=__newr0  mask(Line){p3_4_5q=[32  33  50], p6q=0, p8q=0.0936, p9q=0.209, p10q=0, p13_14_15q=[0.0  0.0  0.0], p16q=on}
      mask prompts: p3_4_5q "Power, Voltage and Frequency Ratings [MVA, kV, Hz]"; p6q "Length of line [km] (0 for p.u. parameters)"; p8q "Resistance [p.u. (Ohms/km)]"; p9q "Reactance [p.u. (H/km)]"; p10q "Susceptance [p.u. (F/km)]"; p13_14_15q "Imax, Pmax and Smax [p.u., p.u., p.u.]"; p16q "Connected"
      mask help: This block defines a pi model for a tree phase line.
      mask init:
      | [xp,yp] = fm_draw('pi');
      mask Callback p16q: fm_block
      mask Display:
      | plot([-1  1  1 -1 -1],[-0.2 -0.2 0.2 0.2 -0.2])
      | color('blue')
      | plot(0.35*xp,0.2*yp)
  Line31 : PMComponent  Tag=PSATblock  Description=Power Flow  PhysicalDomain=psatdomain  LeftPortType=p1  RightPortType=p1  LConnTagsString=__newl0  RConnTagsString=__newr0  mask(Line){p3_4_5q=[32  33  50], p6q=0, p8q=0.0324, p9q=0.0845, p10q=0, p13_14_15q=[0.0  0.0  0.0], p16q=on}
      mask prompts: p3_4_5q "Power, Voltage and Frequency Ratings [MVA, kV, Hz]"; p6q "Length of line [km] (0 for p.u. parameters)"; p8q "Resistance [p.u. (Ohms/km)]"; p9q "Reactance [p.u. (H/km)]"; p10q "Susceptance [p.u. (F/km)]"; p13_14_15q "Imax, Pmax and Smax [p.u., p.u., p.u.]"; p16q "Connected"
      mask help: This block defines a pi model for a tree phase line.
      mask init:
      | [xp,yp] = fm_draw('pi');
      mask Callback p16q: fm_block
      mask Display:
      | plot([-1  1  1 -1 -1],[-0.2 -0.2 0.2 0.2 -0.2])
      | color('blue')
      | plot(0.35*xp,0.2*yp)
  Line32 : PMComponent  Tag=PSATblock  Description=Power Flow  PhysicalDomain=psatdomain  LeftPortType=p1  RightPortType=p1  LConnTagsString=__newl0  RConnTagsString=__newr0  mask(Line){p3_4_5q=[32 132 50], p6q=0, p8q=0.0636, p9q=0.2, p10q=0.0428, p13_14_15q=[0.0  0.0  0.0], p16q=on}
      mask prompts: p3_4_5q "Power, Voltage and Frequency Ratings [MVA, kV, Hz]"; p6q "Length of line [km] (0 for p.u. parameters)"; p8q "Resistance [p.u. (Ohms/km)]"; p9q "Reactance [p.u. (H/km)]"; p10q "Susceptance [p.u. (F/km)]"; p13_14_15q "Imax, Pmax and Smax [p.u., p.u., p.u.]"; p16q "Connected"
      mask help: This block defines a pi model for a tree phase line.
      mask init:
      | [xp,yp] = fm_draw('pi');
      mask Callback p16q: fm_block
      mask Display:
      | plot([-1  1  1 -1 -1],[-0.2 -0.2 0.2 0.2 -0.2])
      | color('blue')
      | plot(0.35*xp,0.2*yp)
  Line34 : PMComponent  Tag=PSATblock  Description=Power Flow  PhysicalDomain=psatdomain  LeftPortType=p1  RightPortType=p1  LConnTagsString=__newl0  RConnTagsString=__newr0  mask(Line){p3_4_5q=[32  132  50], p6q=0, p8q=0.012, p9q=0.042, p10q=0.009, p13_14_15q=[0.0  0.0  0.0], p16q=on}
      mask prompts: p3_4_5q "Power, Voltage and Frequency Ratings [MVA, kV, Hz]"; p6q "Length of line [km] (0 for p.u. parameters)"; p8q "Resistance [p.u. (Ohms/km)]"; p9q "Reactance [p.u. (H/km)]"; p10q "Susceptance [p.u. (F/km)]"; p13_14_15q "Imax, Pmax and Smax [p.u., p.u., p.u.]"; p16q "Connected"
      mask help: This block defines a pi model for a tree phase line.
      mask init:
      | [xp,yp] = fm_draw('pi');
      mask Callback p16q: fm_block
      mask Display:
      | plot([-1  1  1 -1 -1],[-0.2 -0.2 0.2 0.2 -0.2])
      | color('blue')
      | plot(0.35*xp,0.2*yp)
  Line37 : PMComponent  Tag=PSATblock  Description=Power Flow  PhysicalDomain=psatdomain  LeftPortType=p1  RightPortType=p1  LConnTagsString=__newl0  RConnTagsString=__newr0  mask(Line){p3_4_5q=[16 33  50], p6q=0, p8q=0.12, p9q=0, p10q=0, p13_14_15q=[0.0  0.0  0.0], p16q=on}
      mask prompts: p3_4_5q "Power, Voltage and Frequency Ratings [MVA, kV, Hz]"; p6q "Length of line [km] (0 for p.u. parameters)"; p8q "Resistance [p.u. (Ohms/km)]"; p9q "Reactance [p.u. (H/km)]"; p10q "Susceptance [p.u. (F/km)]"; p13_14_15q "Imax, Pmax and Smax [p.u., p.u., p.u.]"; p16q "Connected"
      mask help: This block defines a pi model for a tree phase line.
      mask init:
      | [xp,yp] = fm_draw('pi');
      mask Callback p16q: fm_block
      mask Display:
      | plot([-1  1  1 -1 -1],[-0.2 -0.2 0.2 0.2 -0.2])
      | color('blue')
      | plot(0.35*xp,0.2*yp)
  Line38 : PMComponent  Tag=PSATblock  Description=Power Flow  PhysicalDomain=psatdomain  LeftPortType=p1  RightPortType=p1  LConnTagsString=__newl0  RConnTagsString=__newr0  mask(Line){p3_4_5q=[130  132  50], p6q=0, p8q=0.0267, p9q=0.082, p10q=0.017, p13_14_15q=[0.0  0.0  0.0], p16q=on}
      mask prompts: p3_4_5q "Power, Voltage and Frequency Ratings [MVA, kV, Hz]"; p6q "Length of line [km] (0 for p.u. parameters)"; p8q "Resistance [p.u. (Ohms/km)]"; p9q "Reactance [p.u. (H/km)]"; p10q "Susceptance [p.u. (F/km)]"; p13_14_15q "Imax, Pmax and Smax [p.u., p.u., p.u.]"; p16q "Connected"
      mask help: This block defines a pi model for a tree phase line.
      mask init:
      | [xp,yp] = fm_draw('pi');
      mask Callback p16q: fm_block
      mask Display:
      | plot([-1  1  1 -1 -1],[-0.2 -0.2 0.2 0.2 -0.2])
      | color('blue')
      | plot(0.35*xp,0.2*yp)
  Line39 : PMComponent  Tag=PSATblock  Description=Power Flow  PhysicalDomain=psatdomain  LeftPortType=p1  RightPortType=p1  LConnTagsString=__newl0  RConnTagsString=__newr0  mask(Line){p3_4_5q=[70  132 50], p6q=0, p8q=0.046, p9q=0.116, p10q=0.0204, p13_14_15q=[0.0  0.0  0.0], p16q=on}
      mask prompts: p3_4_5q "Power, Voltage and Frequency Ratings [MVA, kV, Hz]"; p6q "Length of line [km] (0 for p.u. parameters)"; p8q "Resistance [p.u. (Ohms/km)]"; p9q "Reactance [p.u. (H/km)]"; p10q "Susceptance [p.u. (F/km)]"; p13_14_15q "Imax, Pmax and Smax [p.u., p.u., p.u.]"; p16q "Connected"
      mask help: This block defines a pi model for a tree phase line.
      mask init:
      | [xp,yp] = fm_draw('pi');
      mask Callback p16q: fm_block
      mask Display:
      | plot([-1  1  1 -1 -1],[-0.2 -0.2 0.2 0.2 -0.2])
      | color('blue')
      | plot(0.35*xp,0.2*yp)
  Line4 : PMComponent  Tag=PSATblock  Description=Power Flow  PhysicalDomain=psatdomain  LeftPortType=p1  RightPortType=p1  LConnTagsString=__newl0  RConnTagsString=__newr0  mask(Line){p3_4_5q=[130 132 50], p6q=0, p8q=0.0132, p9q=0.0379, p10q=0.0084, p13_14_15q=[0.0  0.0  0.0], p16q=on}
      mask prompts: p3_4_5q "Power, Voltage and Frequency Ratings [MVA, kV, Hz]"; p6q "Length of line [km] (0 for p.u. parameters)"; p8q "Resistance [p.u. (Ohms/km)]"; p9q "Reactance [p.u. (H/km)]"; p10q "Susceptance [p.u. (F/km)]"; p13_14_15q "Imax, Pmax and Smax [p.u., p.u., p.u.]"; p16q "Connected"
      mask help: This block defines a pi model for a tree phase line.
      mask init:
      | [xp,yp] = fm_draw('pi');
      mask Callback p16q: fm_block
      mask Display:
      | plot([-1  1  1 -1 -1],[-0.2 -0.2 0.2 0.2 -0.2])
      | color('blue')
      | plot(0.35*xp,0.2*yp)
  Line43 : PMComponent  Tag=PSATblock  Description=Power Flow  PhysicalDomain=psatdomain  LeftPortType=p1  RightPortType=p1  LConnTagsString=__newl0  RConnTagsString=__newr0  mask(Line){p3_4_5q=[16  33  50], p6q=0, p8q=0.115, p9q=0.179, p10q=0, p13_14_15q=[0.0  0.0  0.0], p16q=on}
      mask prompts: p3_4_5q "Power, Voltage and Frequency Ratings [MVA, kV, Hz]"; p6q "Length of line [km] (0 for p.u. parameters)"; p8q "Resistance [p.u. (Ohms/km)]"; p9q "Reactance [p.u. (H/km)]"; p10q "Susceptance [p.u. (F/km)]"; p13_14_15q "Imax, Pmax and Smax [p.u., p.u., p.u.]"; p16q "Connected"
      mask help: This block defines a pi model for a tree phase line.
      mask init:
      | [xp,yp] = fm_draw('pi');
      mask Callback p16q: fm_block
      mask Display:
      | plot([-1  1  1 -1 -1],[-0.2 -0.2 0.2 0.2 -0.2])
      | color('blue')
      | plot(0.35*xp,0.2*yp)
  Line44 : PMComponent  Tag=PSATblock  Description=Power Flow  PhysicalDomain=psatdomain  LeftPortType=p1  RightPortType=p1  LConnTagsString=__newl0  RConnTagsString=__newr0  mask(Line){p3_4_5q=[16 33 50], p6q=0, p8q=0.080, p9q=0.150, p10q=0, p13_14_15q=[0.0  0.0  0.0], p16q=on}
      mask prompts: p3_4_5q "Power, Voltage and Frequency Ratings [MVA, kV, Hz]"; p6q "Length of line [km] (0 for p.u. parameters)"; p8q "Resistance [p.u. (Ohms/km)]"; p9q "Reactance [p.u. (H/km)]"; p10q "Susceptance [p.u. (F/km)]"; p13_14_15q "Imax, Pmax and Smax [p.u., p.u., p.u.]"; p16q "Connected"
      mask help: This block defines a pi model for a tree phase line.
      mask init:
      | [xp,yp] = fm_draw('pi');
      mask Callback p16q: fm_block
      mask Display:
      | plot([-1  1  1 -1 -1],[-0.2 -0.2 0.2 0.2 -0.2])
      | color('blue')
      | plot(0.35*xp,0.2*yp)
  Line45 : PMComponent  Tag=PSATblock  Description=Power Flow  PhysicalDomain=psatdomain  LeftPortType=p1  RightPortType=p1  LConnTagsString=__newl0  RConnTagsString=__newr0  mask(Line){p3_4_5q=[16 33 50], p6q=0, p8q=0.050, p9q=0.156, p10q=0, p13_14_15q=[0.0  0.0  0.0], p16q=on}
      mask prompts: p3_4_5q "Power, Voltage and Frequency Ratings [MVA, kV, Hz]"; p6q "Length of line [km] (0 for p.u. parameters)"; p8q "Resistance [p.u. (Ohms/km)]"; p9q "Reactance [p.u. (H/km)]"; p10q "Susceptance [p.u. (F/km)]"; p13_14_15q "Imax, Pmax and Smax [p.u., p.u., p.u.]"; p16q "Connected"
      mask help: This block defines a pi model for a tree phase line.
      mask init:
      | [xp,yp] = fm_draw('pi');
      mask Callback p16q: fm_block
      mask Display:
      | plot([-1  1  1 -1 -1],[-0.2 -0.2 0.2 0.2 -0.2])
      | color('blue')
      | plot(0.35*xp,0.2*yp)
  Line46 : PMComponent  Tag=PSATblock  Description=Power Flow  PhysicalDomain=psatdomain  LeftPortType=p1  RightPortType=p1  LConnTagsString=__newl0  RConnTagsString=__newr0  mask(Line){p3_4_5q=[16 33 50], p6q=0, p8q=0.100, p9q=0.352, p10q=0, p13_14_15q=[0.0  0.0  0.0], p16q=on}
      mask prompts: p3_4_5q "Power, Voltage and Frequency Ratings [MVA, kV, Hz]"; p6q "Length of line [km] (0 for p.u. parameters)"; p8q "Resistance [p.u. (Ohms/km)]"; p9q "Reactance [p.u. (H/km)]"; p10q "Susceptance [p.u. (F/km)]"; p13_14_15q "Imax, Pmax and Smax [p.u., p.u., p.u.]"; p16q "Connected"
      mask help: This block defines a pi model for a tree phase line.
      mask init:
      | [xp,yp] = fm_draw('pi');
      mask Callback p16q: fm_block
      mask Display:
      | plot([-1  1  1 -1 -1],[-0.2 -0.2 0.2 0.2 -0.2])
      | color('blue')
      | plot(0.35*xp,0.2*yp)
  Line47 : PMComponent  Tag=PSATblock  Description=Power Flow  PhysicalDomain=psatdomain  LeftPortType=p1  RightPortType=p1  LConnTagsString=__newl0  RConnTagsString=__newr0  mask(Line){p3_4_5q=[16 33 50], p6q=0, p8q=0.05, p9q=0.10, p10q=0, p13_14_15q=[0.0  0.0  0.0], p16q=on}
      mask prompts: p3_4_5q "Power, Voltage and Frequency Ratings [MVA, kV, Hz]"; p6q "Length of line [km] (0 for p.u. parameters)"; p8q "Resistance [p.u. (Ohms/km)]"; p9q "Reactance [p.u. (H/km)]"; p10q "Susceptance [p.u. (F/km)]"; p13_14_15q "Imax, Pmax and Smax [p.u., p.u., p.u.]"; p16q "Connected"
      mask help: This block defines a pi model for a tree phase line.
      mask init:
      | [xp,yp] = fm_draw('pi');
      mask Callback p16q: fm_block
      mask Display:
      | plot([-1  1  1 -1 -1],[-0.2 -0.2 0.2 0.2 -0.2])
      | color('blue')
      | plot(0.35*xp,0.2*yp)
  Line48 : PMComponent  Tag=PSATblock  Description=Power Flow  PhysicalDomain=psatdomain  LeftPortType=p1  RightPortType=p1  LConnTagsString=__newl0  RConnTagsString=__newr0  mask(Line){p3_4_5q=[16  33  50], p6q=0, p8q=0.05, p9q=0.10, p10q=0, p13_14_15q=[0.0  0.0  0.0], p16q=on}
      mask prompts: p3_4_5q "Power, Voltage and Frequency Ratings [MVA, kV, Hz]"; p6q "Length of line [km] (0 for p.u. parameters)"; p8q "Resistance [p.u. (Ohms/km)]"; p9q "Reactance [p.u. (H/km)]"; p10q "Susceptance [p.u. (F/km)]"; p13_14_15q "Imax, Pmax and Smax [p.u., p.u., p.u.]"; p16q "Connected"
      mask help: This block defines a pi model for a tree phase line.
      mask init:
      | [xp,yp] = fm_draw('pi');
      mask Callback p16q: fm_block
      mask Display:
      | plot([-1  1  1 -1 -1],[-0.2 -0.2 0.2 0.2 -0.2])
      | color('blue')
      | plot(0.35*xp,0.2*yp)
  Line5 : PMComponent  Tag=PSATblock  Description=Power Flow  PhysicalDomain=psatdomain  LeftPortType=p1  RightPortType=p1  LConnTagsString=__newl0  RConnTagsString=__newr0  mask(Line){p3_4_5q=[100  11  50], p6q=0, p8q=0, p9q=0.14, p10q=0, p13_14_15q=[0.0  0.0  0.0], p16q=on}
      mask prompts: p3_4_5q "Power, Voltage and Frequency Ratings [MVA, kV, Hz]"; p6q "Length of line [km] (0 for p.u. parameters)"; p8q "Resistance [p.u. (Ohms/km)]"; p9q "Reactance [p.u. (H/km)]"; p10q "Susceptance [p.u. (F/km)]"; p13_14_15q "Imax, Pmax and Smax [p.u., p.u., p.u.]"; p16q "Connected"
      mask help: This block defines a pi model for a tree phase line.
      mask init:
      | [xp,yp] = fm_draw('pi');
      mask Callback p16q: fm_block
      mask Display:
      | plot([-1  1  1 -1 -1],[-0.2 -0.2 0.2 0.2 -0.2])
      | color('blue')
      | plot(0.35*xp,0.2*yp)
  Line6 : PMComponent  Tag=PSATblock  Description=Power Flow  PhysicalDomain=psatdomain  LeftPortType=p1  RightPortType=p1  LConnTagsString=__newl0  RConnTagsString=__newr0  mask(Line){p3_4_5q=[100  132  50], p6q=0, p8q=0, p9q=0.208, p10q=0, p13_14_15q=[0.0  0.0  0.0], p16q=on}
      mask prompts: p3_4_5q "Power, Voltage and Frequency Ratings [MVA, kV, Hz]"; p6q "Length of line [km] (0 for p.u. parameters)"; p8q "Resistance [p.u. (Ohms/km)]"; p9q "Reactance [p.u. (H/km)]"; p10q "Susceptance [p.u. (F/km)]"; p13_14_15q "Imax, Pmax and Smax [p.u., p.u., p.u.]"; p16q "Connected"
      mask help: This block defines a pi model for a tree phase line.
      mask init:
      | [xp,yp] = fm_draw('pi');
      mask Callback p16q: fm_block
      mask Display:
      | plot([-1  1  1 -1 -1],[-0.2 -0.2 0.2 0.2 -0.2])
      | color('blue')
      | plot(0.35*xp,0.2*yp)
  Line7 : PMComponent  Tag=PSATblock  Description=Power Flow  PhysicalDomain=psatdomain  LeftPortType=p1  RightPortType=p1  LConnTagsString=__newl0  RConnTagsString=__newr0  mask(Line){p3_4_5q=[130  132 50], p6q=0, p8q=0.0192, p9q=0.0575, p10q=0.0528, p13_14_15q=[0.0  0.0  0.0], p16q=on}
      mask prompts: p3_4_5q "Power, Voltage and Frequency Ratings [MVA, kV, Hz]"; p6q "Length of line [km] (0 for p.u. parameters)"; p8q "Resistance [p.u. (Ohms/km)]"; p9q "Reactance [p.u. (H/km)]"; p10q "Susceptance [p.u. (F/km)]"; p13_14_15q "Imax, Pmax and Smax [p.u., p.u., p.u.]"; p16q "Connected"
      mask help: This block defines a pi model for a tree phase line.
      mask init:
      | [xp,yp] = fm_draw('pi');
      mask Callback p16q: fm_block
      mask Display:
      | plot([-1  1  1 -1 -1],[-0.2 -0.2 0.2 0.2 -0.2])
      | color('blue')
      | plot(0.35*xp,0.2*yp)
  Line8 : PMComponent  Tag=PSATblock  Description=Power Flow  PhysicalDomain=psatdomain  LeftPortType=p1  RightPortType=p1  LConnTagsString=__newl0  RConnTagsString=__newr0  mask(Line){p3_4_5q=[100  1  50], p6q=0, p8q=0, p9q=0.208, p10q=0, p13_14_15q=[0.0  0.0  0.0], p16q=on}
      mask prompts: p3_4_5q "Power, Voltage and Frequency Ratings [MVA, kV, Hz]"; p6q "Length of line [km] (0 for p.u. parameters)"; p8q "Resistance [p.u. (Ohms/km)]"; p9q "Reactance [p.u. (H/km)]"; p10q "Susceptance [p.u. (F/km)]"; p13_14_15q "Imax, Pmax and Smax [p.u., p.u., p.u.]"; p16q "Connected"
      mask help: This block defines a pi model for a tree phase line.
      mask init:
      | [xp,yp] = fm_draw('pi');
      mask Callback p16q: fm_block
      mask Display:
      | plot([-1  1  1 -1 -1],[-0.2 -0.2 0.2 0.2 -0.2])
      | color('blue')
      | plot(0.35*xp,0.2*yp)
  Line9 : PMComponent  Tag=PSATblock  Description=Power Flow  PhysicalDomain=psatdomain  LeftPortType=p1  RightPortType=p1  LConnTagsString=__newl0  RConnTagsString=__newr0  mask(Line){p3_4_5q=[100  1  50], p6q=0, p8q=0, p9q=0.11, p10q=0, p13_14_15q=[0.0  0.0  0.0], p16q=on}
      mask prompts: p3_4_5q "Power, Voltage and Frequency Ratings [MVA, kV, Hz]"; p6q "Length of line [km] (0 for p.u. parameters)"; p8q "Resistance [p.u. (Ohms/km)]"; p9q "Reactance [p.u. (H/km)]"; p10q "Susceptance [p.u. (F/km)]"; p13_14_15q "Imax, Pmax and Smax [p.u., p.u., p.u.]"; p16q "Connected"
      mask help: This block defines a pi model for a tree phase line.
      mask init:
      | [xp,yp] = fm_draw('pi');
      mask Callback p16q: fm_block
      mask Display:
      | plot([-1  1  1 -1 -1],[-0.2 -0.2 0.2 0.2 -0.2])
      | color('blue')
      | plot(0.35*xp,0.2*yp)
  PQ : PMComponent  Tag=PSATblock  Description=Power Flow  PhysicalDomain=psatdomain  LeftPortType=p1  RightPortType=p1  LConnTagsString=__newl0  mask(PQ){p2_3q=[100  132], p4_5q=[0.217  0.127], p6_7q=[0.5  -0.4], p8q=off, p9q=on}
      mask prompts: p2_3q "Power and Voltage Ratings [MVA, kV]"; p4_5q "Active and Reactive Powers [p.u.  p.u.]"; p6_7q "Maximum and Minimum Allowable Voltage [p.u.   p.u.]"; p8q "Allow conversion to impendance for min or max voltage"; p9q "Connected"
      mask help:
      | This block defines a constant power load:
      |
      | P = Pcost.
      | Q = Qcost.
      mask Callback p8q: fm_block
      mask Callback p9q: fm_block
      mask Display: plot([1 -0.5 -0.5 1],[0 0.866 -0.866 0])
  PQ1 : PMComponent  Tag=PSATblock  Description=Power Flow  PhysicalDomain=psatdomain  LeftPortType=p1  RightPortType=p1  LConnTagsString=__newl0  mask(PQ){p2_3q=[100  132], p4_5q=[0.30  0.30], p6_7q=[1.2  0.8], p8q=off, p9q=on}
      mask prompts: p2_3q "Power and Voltage Ratings [MVA, kV]"; p4_5q "Active and Reactive Powers [p.u.  p.u.]"; p6_7q "Maximum and Minimum Allowable Voltage [p.u.   p.u.]"; p8q "Allow conversion to impendance for min or max voltage"; p9q "Connected"
      mask help:
      | This block defines a constant power load:
      |
      | P = Pcost.
      | Q = Qcost.
      mask Callback p8q: fm_block
      mask Callback p9q: fm_block
      mask Display: plot([1 -0.5 -0.5 1],[0 0.866 -0.866 0])
  PQ11 : PMComponent  Tag=PSATblock  Description=Power Flow  PhysicalDomain=psatdomain  LeftPortType=p1  RightPortType=p1  LConnTagsString=__newl0  mask(PQ){p2_3q=[100  33], p4_5q=[0.075  0.015], p6_7q=[0  0], p8q=on, p9q=on}
      mask prompts: p2_3q "Power and Voltage Ratings [MVA, kV]"; p4_5q "Active and Reactive Powers [p.u.  p.u.]"; p6_7q "Maximum and Minimum Allowable Voltage [p.u.   p.u.]"; p8q "Allow conversion to impendance for min or max voltage"; p9q "Connected"
      mask help:
      | This block defines a constant power load:
      |
      | P = Pcost.
      | Q = Qcost.
      mask Callback p8q: fm_block
      mask Callback p9q: fm_block
      mask Display: plot([1 -0.5 -0.5 1],[0 0.866 -0.866 0])
  PQ14 : PMComponent  Tag=PSATblock  Description=Power Flow  PhysicalDomain=psatdomain  LeftPortType=p1  RightPortType=p1  LConnTagsString=__newl0  mask(PQ){p2_3q=[100  132], p4_5q=[0.942  0.19], p6_7q=[0.4  -0.4], p8q=off, p9q=on}
      mask prompts: p2_3q "Power and Voltage Ratings [MVA, kV]"; p4_5q "Active and Reactive Powers [p.u.  p.u.]"; p6_7q "Maximum and Minimum Allowable Voltage [p.u.   p.u.]"; p8q "Allow conversion to impendance for min or max voltage"; p9q "Connected"
      mask help:
      | This block defines a constant power load:
      |
      | P = Pcost.
      | Q = Qcost.
      mask Callback p8q: fm_block
      mask Callback p9q: fm_block
      mask Display: plot([1 -0.5 -0.5 1],[0 0.866 -0.866 0])
  PQ15 : PMComponent  Tag=PSATblock  Description=Power Flow  PhysicalDomain=psatdomain  LeftPortType=p1  RightPortType=p1  LConnTagsString=__newl0  mask(PQ){p2_3q=[100  33], p4_5q=[0.032  0.016], p6_7q=[0  0.0], p8q=off, p9q=on}
      mask prompts: p2_3q "Power and Voltage Ratings [MVA, kV]"; p4_5q "Active and Reactive Powers [p.u.  p.u.]"; p6_7q "Maximum and Minimum Allowable Voltage [p.u.   p.u.]"; p8q "Allow conversion to impendance for min or max voltage"; p9q "Connected"
      mask help:
      | This block defines a constant power load:
      |
      | P = Pcost.
      | Q = Qcost.
      mask Callback p8q: fm_block
      mask Callback p9q: fm_block
      mask Display: plot([1 -0.5 -0.5 1],[0 0.866 -0.866 0])
  PQ16 : PMComponent  Tag=PSATblock  Description=Power Flow  PhysicalDomain=psatdomain  LeftPortType=p1  RightPortType=p1  LConnTagsString=__newl0  mask(PQ){p2_3q=[100  132], p4_5q=[0.228 0.109], p6_7q=[0  0], p8q=off, p9q=on}
      mask prompts: p2_3q "Power and Voltage Ratings [MVA, kV]"; p4_5q "Active and Reactive Powers [p.u.  p.u.]"; p6_7q "Maximum and Minimum Allowable Voltage [p.u.   p.u.]"; p8q "Allow conversion to impendance for min or max voltage"; p9q "Connected"
      mask help:
      | This block defines a constant power load:
      |
      | P = Pcost.
      | Q = Qcost.
      mask Callback p8q: fm_block
      mask Callback p9q: fm_block
      mask Display: plot([1 -0.5 -0.5 1],[0 0.866 -0.866 0])
  PQ17 : PMComponent  Tag=PSATblock  Description=Power Flow  PhysicalDomain=psatdomain  LeftPortType=p1  RightPortType=p1  LConnTagsString=__newl0  mask(PQ){p2_3q=[100  33], p4_5q=[0.09  0.058], p6_7q=[0  0], p8q=off, p9q=on}
      mask prompts: p2_3q "Power and Voltage Ratings [MVA, kV]"; p4_5q "Active and Reactive Powers [p.u.  p.u.]"; p6_7q "Maximum and Minimum Allowable Voltage [p.u.   p.u.]"; p8q "Allow conversion to impendance for min or max voltage"; p9q "Connected"
      mask help:
      | This block defines a constant power load:
      |
      | P = Pcost.
      | Q = Qcost.
      mask Callback p8q: fm_block
      mask Callback p9q: fm_block
      mask Display: plot([1 -0.5 -0.5 1],[0 0.866 -0.866 0])
  PQ18 : PMComponent  Tag=PSATblock  Description=Power Flow  PhysicalDomain=psatdomain  LeftPortType=p1  RightPortType=p1  LConnTagsString=__newl0  mask(PQ){p2_3q=[100  33], p4_5q=[0.025  0.013], p6_7q=[0  0], p8q=off, p9q=on}
      mask prompts: p2_3q "Power and Voltage Ratings [MVA, kV]"; p4_5q "Active and Reactive Powers [p.u.  p.u.]"; p6_7q "Maximum and Minimum Allowable Voltage [p.u.   p.u.]"; p8q "Allow conversion to impendance for min or max voltage"; p9q "Connected"
      mask help:
      | This block defines a constant power load:
      |
      | P = Pcost.
      | Q = Qcost.
      mask Callback p8q: fm_block
      mask Callback p9q: fm_block
      mask Display: plot([1 -0.5 -0.5 1],[0 0.866 -0.866 0])
  PQ19 : PMComponent  Tag=PSATblock  Description=Power Flow  PhysicalDomain=psatdomain  LeftPortType=p1  RightPortType=p1  LConnTagsString=__newl0  mask(PQ){p2_3q=[100  132], p4_5q=[0.024 0.012], p6_7q=[0 0], p8q=off, p9q=on}
      mask prompts: p2_3q "Power and Voltage Ratings [MVA, kV]"; p4_5q "Active and Reactive Powers [p.u.  p.u.]"; p6_7q "Maximum and Minimum Allowable Voltage [p.u.   p.u.]"; p8q "Allow conversion to impendance for min or max voltage"; p9q "Connected"
      mask help:
      | This block defines a constant power load:
      |
      | P = Pcost.
      | Q = Qcost.
      mask Callback p8q: fm_block
      mask Callback p9q: fm_block
      mask Display: plot([1 -0.5 -0.5 1],[0 0.866 -0.866 0])
  PQ2 : PMComponent  Tag=PSATblock  Description=Power Flow  PhysicalDomain=psatdomain  LeftPortType=p1  RightPortType=p1  LConnTagsString=__newl0  mask(PQ){p2_3q=[100  33], p4_5q=[0.087  0.067], p6_7q=[0  0], p8q=on, p9q=on}
      mask prompts: p2_3q "Power and Voltage Ratings [MVA, kV]"; p4_5q "Active and Reactive Powers [p.u.  p.u.]"; p6_7q "Maximum and Minimum Allowable Voltage [p.u.   p.u.]"; p8q "Allow conversion to impendance for min or max voltage"; p9q "Connected"
      mask help:
      | This block defines a constant power load:
      |
      | P = Pcost.
      | Q = Qcost.
      mask Callback p8q: fm_block
      mask Callback p9q: fm_block
      mask Display: plot([1 -0.5 -0.5 1],[0 0.866 -0.866 0])
  PQ21 : PMComponent  Tag=PSATblock  Description=Power Flow  PhysicalDomain=psatdomain  LeftPortType=p1  RightPortType=p1  LConnTagsString=__newl0  mask(PQ){p2_3q=[100  33], p4_5q=[.112 0.075], p6_7q=[0 0], p8q=off, p9q=on}
      mask prompts: p2_3q "Power and Voltage Ratings [MVA, kV]"; p4_5q "Active and Reactive Powers [p.u.  p.u.]"; p6_7q "Maximum and Minimum Allowable Voltage [p.u.   p.u.]"; p8q "Allow conversion to impendance for min or max voltage"; p9q "Connected"
      mask help:
      | This block defines a constant power load:
      |
      | P = Pcost.
      | Q = Qcost.
      mask Callback p8q: fm_block
      mask Callback p9q: fm_block
      mask Display: plot([1 -0.5 -0.5 1],[0 0.866 -0.866 0])
  PQ22 : PMComponent  Tag=PSATblock  Description=Power Flow  PhysicalDomain=psatdomain  LeftPortType=p1  RightPortType=p1  LConnTagsString=__newl0  mask(PQ){p2_3q=[100  33], p4_5q=[0.062  0.016], p6_7q=[0 0], p8q=off, p9q=on}
      mask prompts: p2_3q "Power and Voltage Ratings [MVA, kV]"; p4_5q "Active and Reactive Powers [p.u.  p.u.]"; p6_7q "Maximum and Minimum Allowable Voltage [p.u.   p.u.]"; p8q "Allow conversion to impendance for min or max voltage"; p9q "Connected"
      mask help:
      | This block defines a constant power load:
      |
      | P = Pcost.
      | Q = Qcost.
      mask Callback p8q: fm_block
      mask Callback p9q: fm_block
      mask Display: plot([1 -0.5 -0.5 1],[0 0.866 -0.866 0])
  PQ23 : PMComponent  Tag=PSATblock  Description=Power Flow  PhysicalDomain=psatdomain  LeftPortType=p1  RightPortType=p1  LConnTagsString=__newl0  mask(PQ){p2_3q=[100  33], p4_5q=[0.082 0.025], p6_7q=[0 0], p8q=off, p9q=on}
      mask prompts: p2_3q "Power and Voltage Ratings [MVA, kV]"; p4_5q "Active and Reactive Powers [p.u.  p.u.]"; p6_7q "Maximum and Minimum Allowable Voltage [p.u.   p.u.]"; p8q "Allow conversion to impendance for min or max voltage"; p9q "Connected"
      mask help:
      | This block defines a constant power load:
      |
      | P = Pcost.
      | Q = Qcost.
      mask Callback p8q: fm_block
      mask Callback p9q: fm_block
      mask Display: plot([1 -0.5 -0.5 1],[0 0.866 -0.866 0])
  PQ24 : PMComponent  Tag=PSATblock  Description=Power Flow  PhysicalDomain=psatdomain  LeftPortType=p1  RightPortType=p1  LConnTagsString=__newl0  mask(PQ){p2_3q=[100  33], p4_5q=[0.035 0.018], p6_7q=[0  0], p8q=off, p9q=on}
      mask prompts: p2_3q "Power and Voltage Ratings [MVA, kV]"; p4_5q "Active and Reactive Powers [p.u.  p.u.]"; p6_7q "Maximum and Minimum Allowable Voltage [p.u.   p.u.]"; p8q "Allow conversion to impendance for min or max voltage"; p9q "Connected"
      mask help:
      | This block defines a constant power load:
      |
      | P = Pcost.
      | Q = Qcost.
      mask Callback p8q: fm_block
      mask Callback p9q: fm_block
      mask Display: plot([1 -0.5 -0.5 1],[0 0.866 -0.866 0])
  PQ25 : PMComponent  Tag=PSATblock  Description=Power Flow  PhysicalDomain=psatdomain  LeftPortType=p1  RightPortType=p1  LConnTagsString=__newl0  mask(PQ){p2_3q=[100  33], p4_5q=[0.032  0.009], p6_7q=[0 0], p8q=off, p9q=on}
      mask prompts: p2_3q "Power and Voltage Ratings [MVA, kV]"; p4_5q "Active and Reactive Powers [p.u.  p.u.]"; p6_7q "Maximum and Minimum Allowable Voltage [p.u.   p.u.]"; p8q "Allow conversion to impendance for min or max voltage"; p9q "Connected"
      mask help:
      | This block defines a constant power load:
      |
      | P = Pcost.
      | Q = Qcost.
      mask Callback p8q: fm_block
      mask Callback p9q: fm_block
      mask Display: plot([1 -0.5 -0.5 1],[0 0.866 -0.866 0])
  PQ26 : PMComponent  Tag=PSATblock  Description=Power Flow  PhysicalDomain=psatdomain  LeftPortType=p1  RightPortType=p1  LConnTagsString=__newl0  mask(PQ){p2_3q=[100 33], p4_5q=[0.022  0.007], p6_7q=[1.2  0.8], p8q=off, p9q=on}
      mask prompts: p2_3q "Power and Voltage Ratings [MVA, kV]"; p4_5q "Active and Reactive Powers [p.u.  p.u.]"; p6_7q "Maximum and Minimum Allowable Voltage [p.u.   p.u.]"; p8q "Allow conversion to impendance for min or max voltage"; p9q "Connected"
      mask help:
      | This block defines a constant power load:
      |
      | P = Pcost.
      | Q = Qcost.
      mask Callback p8q: fm_block
      mask Callback p9q: fm_block
      mask Display: plot([1 -0.5 -0.5 1],[0 0.866 -0.866 0])
  PQ27 : PMComponent  Tag=PSATblock  Description=Power Flow  PhysicalDomain=psatdomain  LeftPortType=p1  RightPortType=p1  LConnTagsString=__newl0  mask(PQ){p2_3q=[100  33], p4_5q=[0.020  0.009], p6_7q=[0  0], p8q=off, p9q=on}
      mask prompts: p2_3q "Power and Voltage Ratings [MVA, kV]"; p4_5q "Active and Reactive Powers [p.u.  p.u.]"; p6_7q "Maximum and Minimum Allowable Voltage [p.u.   p.u.]"; p8q "Allow conversion to impendance for min or max voltage"; p9q "Connected"
      mask help:
      | This block defines a constant power load:
      |
      | P = Pcost.
      | Q = Qcost.
      mask Callback p8q: fm_block
      mask Callback p9q: fm_block
      mask Display: plot([1 -0.5 -0.5 1],[0 0.866 -0.866 0])
  PQ3 : PMComponent  Tag=PSATblock  Description=Power Flow  PhysicalDomain=psatdomain  LeftPortType=p1  RightPortType=p1  LConnTagsString=__newl0  mask(PQ){p2_3q=[100  33], p4_5q=[0.175  0.112], p6_7q=[0  0], p8q=off, p9q=on}
      mask prompts: p2_3q "Power and Voltage Ratings [MVA, kV]"; p4_5q "Active and Reactive Powers [p.u.  p.u.]"; p6_7q "Maximum and Minimum Allowable Voltage [p.u.   p.u.]"; p8q "Allow conversion to impendance for min or max voltage"; p9q "Connected"
      mask help:
      | This block defines a constant power load:
      |
      | P = Pcost.
      | Q = Qcost.
      mask Callback p8q: fm_block
      mask Callback p9q: fm_block
      mask Display: plot([1 -0.5 -0.5 1],[0 0.866 -0.866 0])
  PQ4 : PMComponent  Tag=PSATblock  Description=Power Flow  PhysicalDomain=psatdomain  LeftPortType=p1  RightPortType=p1  LConnTagsString=__newl0  mask(PQ){p2_3q=[100  132], p4_5q=[0.076  0.016], p6_7q=[0 0], p8q=on, p9q=on}
      mask prompts: p2_3q "Power and Voltage Ratings [MVA, kV]"; p4_5q "Active and Reactive Powers [p.u.  p.u.]"; p6_7q "Maximum and Minimum Allowable Voltage [p.u.   p.u.]"; p8q "Allow conversion to impendance for min or max voltage"; p9q "Connected"
      mask help:
      | This block defines a constant power load:
      |
      | P = Pcost.
      | Q = Qcost.
      mask Callback p8q: fm_block
      mask Callback p9q: fm_block
      mask Display: plot([1 -0.5 -0.5 1],[0 0.866 -0.866 0])
  PQ5 : PMComponent  Tag=PSATblock  Description=Power Flow  PhysicalDomain=psatdomain  LeftPortType=p1  RightPortType=p1  LConnTagsString=__newl0  mask(PQ){p2_3q=[100  33], p4_5q=[0.058  0.02], p6_7q=[0 0], p8q=off, p9q=on}
      mask prompts: p2_3q "Power and Voltage Ratings [MVA, kV]"; p4_5q "Active and Reactive Powers [p.u.  p.u.]"; p6_7q "Maximum and Minimum Allowable Voltage [p.u.   p.u.]"; p8q "Allow conversion to impendance for min or max voltage"; p9q "Connected"
      mask help:
      | This block defines a constant power load:
      |
      | P = Pcost.
      | Q = Qcost.
      mask Callback p8q: fm_block
      mask Callback p9q: fm_block
      mask Display: plot([1 -0.5 -0.5 1],[0 0.866 -0.866 0])
  PQ6 : PMComponent  Tag=PSATblock  Description=Power Flow  PhysicalDomain=psatdomain  LeftPortType=p1  RightPortType=p1  LConnTagsString=__newl0  mask(PQ){p2_3q=[100  33], p4_5q=[0.095  0.034], p6_7q=[1.2  0.8], p8q=off, p9q=on}
      mask prompts: p2_3q "Power and Voltage Ratings [MVA, kV]"; p4_5q "Active and Reactive Powers [p.u.  p.u.]"; p6_7q "Maximum and Minimum Allowable Voltage [p.u.   p.u.]"; p8q "Allow conversion to impendance for min or max voltage"; p9q "Connected"
      mask help:
      | This block defines a constant power load:
      |
      | P = Pcost.
      | Q = Qcost.
      mask Callback p8q: fm_block
      mask Callback p9q: fm_block
      mask Display: plot([1 -0.5 -0.5 1],[0 0.866 -0.866 0])
  PV : PMComponent  Tag=PSATblock  Description=Power Flow  PhysicalDomain=psatdomain  LeftPortType=p1  RightPortType=p1  RConnTagsString=__newr0  mask(PV){p2_3q=[100  132], p4q=.20, p5q=1.045, p6_7q=[1.0 -.20], p8_9q=[1.1  0.9], p10q=1, p11q=on}
      mask prompts: p2_3q "Power and Voltage Ratings [MVA, kV]"; p4q "Active Power [p.u.]"; p5q "Voltage Magnitude [p.u.]"; p6_7q "Qmax and Qmin [p.u.  p.u.]"; p8_9q "Vmax and Vmin [p.u.  p.u.]"; p10q "Loss Participation Factor"; p11q "Connected"
      mask help:
      | This block defines a PV bus for load flow studies:
      |
      | P = Pcost.
      | V = Vdes.
      mask init:
      | [x,y] = fm_draw('circle');
      | [xp,yp] = fm_draw('P');
      mask Callback p11q: fm_block
      mask Display:
      | plot(x,y)
      | color('blue')
      | plot(0.3*xp-0.35,0.6*yp,[0.1 0.3 0.5],[0.3 -0.3 0.3])
  PV1 : PMComponent  Tag=PSATblock  Description=Power Flow  PhysicalDomain=psatdomain  LeftPortType=p1  RightPortType=p1  RConnTagsString=__newr0  mask(PV){p2_3q=[100  132], p4q=.15, p5q=1.01, p6_7q=[.80 -.15], p8_9q=[1.1  0.9], p10q=1, p11q=on}
      mask prompts: p2_3q "Power and Voltage Ratings [MVA, kV]"; p4q "Active Power [p.u.]"; p5q "Voltage Magnitude [p.u.]"; p6_7q "Qmax and Qmin [p.u.  p.u.]"; p8_9q "Vmax and Vmin [p.u.  p.u.]"; p10q "Loss Participation Factor"; p11q "Connected"
      mask help:
      | This block defines a PV bus for load flow studies:
      |
      | P = Pcost.
      | V = Vdes.
      mask init:
      | [x,y] = fm_draw('circle');
      | [xp,yp] = fm_draw('P');
      mask Callback p11q: fm_block
      mask Display:
      | plot(x,y)
      | color('blue')
      | plot(0.3*xp-0.35,0.6*yp,[0.1 0.3 0.5],[0.3 -0.3 0.3])
  PV2 : PMComponent  Tag=PSATblock  Description=Power Flow  PhysicalDomain=psatdomain  LeftPortType=p1  RightPortType=p1  RConnTagsString=__newr0  mask(PV){p2_3q=[100  132], p4q=.10, p5q=1.00, p6_7q=[.60 -.15], p8_9q=[1.1  0.9], p10q=1, p11q=on}
      mask prompts: p2_3q "Power and Voltage Ratings [MVA, kV]"; p4q "Active Power [p.u.]"; p5q "Voltage Magnitude [p.u.]"; p6_7q "Qmax and Qmin [p.u.  p.u.]"; p8_9q "Vmax and Vmin [p.u.  p.u.]"; p10q "Loss Participation Factor"; p11q "Connected"
      mask help:
      | This block defines a PV bus for load flow studies:
      |
      | P = Pcost.
      | V = Vdes.
      mask init:
      | [x,y] = fm_draw('circle');
      | [xp,yp] = fm_draw('P');
      mask Callback p11q: fm_block
      mask Display:
      | plot(x,y)
      | color('blue')
      | plot(0.3*xp-0.35,0.6*yp,[0.1 0.3 0.5],[0.3 -0.3 0.3])
  PV3 : PMComponent  Tag=PSATblock  Description=Power Flow  PhysicalDomain=psatdomain  LeftPortType=p1  RightPortType=p1  RConnTagsString=__newr0  mask(PV){p2_3q=[100  132], p4q=.10, p5q=1.082, p6_7q=[.60 -.15], p8_9q=[1.1  0.9], p10q=1, p11q=on}
      mask prompts: p2_3q "Power and Voltage Ratings [MVA, kV]"; p4q "Active Power [p.u.]"; p5q "Voltage Magnitude [p.u.]"; p6_7q "Qmax and Qmin [p.u.  p.u.]"; p8_9q "Vmax and Vmin [p.u.  p.u.]"; p10q "Loss Participation Factor"; p11q "Connected"
      mask help:
      | This block defines a PV bus for load flow studies:
      |
      | P = Pcost.
      | V = Vdes.
      mask init:
      | [x,y] = fm_draw('circle');
      | [xp,yp] = fm_draw('P');
      mask Callback p11q: fm_block
      mask Display:
      | plot(x,y)
      | color('blue')
      | plot(0.3*xp-0.35,0.6*yp,[0.1 0.3 0.5],[0.3 -0.3 0.3])
  PV4 : PMComponent  Tag=PSATblock  Description=Power Flow  PhysicalDomain=psatdomain  LeftPortType=p1  RightPortType=p1  RConnTagsString=__newr0  mask(PV){p2_3q=[100  11], p4q=0.12, p5q=1.071, p6_7q=[.60 -.15], p8_9q=[1.1  0.9], p10q=1, p11q=on}
      mask prompts: p2_3q "Power and Voltage Ratings [MVA, kV]"; p4q "Active Power [p.u.]"; p5q "Voltage Magnitude [p.u.]"; p6_7q "Qmax and Qmin [p.u.  p.u.]"; p8_9q "Vmax and Vmin [p.u.  p.u.]"; p10q "Loss Participation Factor"; p11q "Connected"
      mask help:
      | This block defines a PV bus for load flow studies:
      |
      | P = Pcost.
      | V = Vdes.
      mask init:
      | [x,y] = fm_draw('circle');
      | [xp,yp] = fm_draw('P');
      mask Callback p11q: fm_block
      mask Display:
      | plot(x,y)
      | color('blue')
      | plot(0.3*xp-0.35,0.6*yp,[0.1 0.3 0.5],[0.3 -0.3 0.3])
  Shunt1 : PMComponent  Tag=PSATblock  Description=Power Flow  PhysicalDomain=psatdomain  LeftPortType=p1  RightPortType=p1  LConnTagsString=__newl0  mask(Shunt){p2_3_4q=[100  33  50], p6q=0.19, p7q=on}
      mask prompts: p2_3_4q "Power, Voltage and Frequency Ratings [MVA, kV, Hz]"; p6q "Susceptance B [p.u.]"; p7q "Connected"
      mask help:
      | This block defines a static condenser:
      |
      | Q = B * V^2
      |
      | (Negative values of B define an inductive load).
      mask init:
      | fm_block
      mask Callback p7q: fm_block
      mask Display: plot(-[0 60 60 55 53 55 60 60 55 53]/150,[0 0 8 16 25 16 8 -8 -16 -25]/50,-[80 80 80 150]/150,[25 -25 0 0]/50,[0 0],[-0.4 0.4],[0.075 0.075],[-0.25 0.25],[0.15 0.15],[-0.1 0.1])
  Shunt2 : PMComponent  Tag=PSATblock  Description=Power Flow  PhysicalDomain=psatdomain  LeftPortType=p1  RightPortType=p1  LConnTagsString=__newl0  mask(Shunt){p2_3_4q=[100  32  50], p6q=0.050, p7q=on}
      mask prompts: p2_3_4q "Power, Voltage and Frequency Ratings [MVA, kV, Hz]"; p6q "Susceptance B [p.u.]"; p7q "Connected"
      mask help:
      | This block defines a static condenser:
      |
      | Q = B * V^2
      |
      | (Negative values of B define an inductive load).
      mask init:
      | fm_block
      mask Callback p7q: fm_block
      mask Display: plot(-[0 60 60 55 53 55 60 60 55 53]/150,[0 0 8 16 25 16 8 -8 -16 -25]/50,-[80 80 80 150]/150,[25 -25 0 0]/50,[0 0],[-0.4 0.4],[0.075 0.075],[-0.25 0.25],[0.15 0.15],[-0.1 0.1])
  Slack : PMComponent  Tag=PSATblock  Description=Power Flow  PhysicalDomain=psatdomain  LeftPortType=p1  RightPortType=p1  RConnTagsString=__newr0  mask(SW){p2_3q=[100  132], p4q=1.06, p5q=0.00, p6_7q=[2.50  -.20], p8_9q=[1.1  0.9], p10q=0.50, p11q=1, p12q=on, p13q=on}
      mask prompts: p2_3q "Power and Voltage Ratings [MVA, kV]"; p4q "Voltage Magnitude [p.u.]"; p5q "Reference Phase Angle [rad]"; p6_7q "Qmax and Qmin [p.u.  p.u.]"; p8_9q "Vmax and Vmin  [p.u.  p.u.]"; p10q "Active Power Guess [p.u.]"; p11q "Loss Participation Factor"; p12q "Reference bus"; p13q "Connected"
      mask help:
      | This block defines a V-theta bus:
      |
      | V = V_des
      | theta = theta_des
      mask init:
      | [x,y] = fm_draw('circle');
      | [xt,yt] = fm_draw('theta');
      mask Callback p12q: fm_block
      mask Callback p13q: fm_block
      mask Display: plot([0 1 1 0 0],[0 0 1 1 0]), color('blue'), plot([0 1],[0 1],[0 1],[1 0],[0.5 1 0.5 0 0.5],[0 0.5 1 0.5 0])
  Slack1 : PMComponent  Tag=PSATblock  Description=Power Flow  PhysicalDomain=psatdomain  LeftPortType=blob  RightPortType=blob  RConnTagsString=__newr0  mask(SW){p2_3q=[100  33], p4q=1.00, p5q=0.00, p6_7q=[1.5  -1.5], p8_9q=[1.1  0.9], p10q=0.80, p11q=1, p12q=off, p13q=on}
      mask prompts: p2_3q "Power and Voltage Ratings [MVA, kV]"; p4q "Voltage Magnitude [p.u.]"; p5q "Reference Phase Angle [rad]"; p6_7q "Qmax and Qmin [p.u.  p.u.]"; p8_9q "Vmax and Vmin  [p.u.  p.u.]"; p10q "Active Power Guess [p.u.]"; p11q "Loss Participation Factor"; p12q "Reference bus"; p13q "Connected"
      mask help:
      | This block defines a V-theta bus:
      |
      | V = V_des
      | theta = theta_des
      mask init:
      | [x,y] = fm_draw('circle');
      | [xt,yt] = fm_draw('theta');
      mask Callback p12q: fm_block
      mask Callback p13q: fm_block
      mask Display: plot(x,y), color('blue'), plot([0.1 0.3 0.5]-0.6,[0.3 -0.3 0.3],0.45*xt+0.1,0.6*yt)
  Transf1 : PMComponent  Tag=PSATblock  Description=Power Flow  PhysicalDomain=psatdomain  LeftPortType=p1  RightPortType=p1  LConnTagsString=__newl0  RConnTagsString=__newr0  mask(Line){p3_4_5q=[32  132  50], p7q=132/33, p8q=0, p9q=0.556, p11q=0.962, p13_14_15q=[0.0  0.0  0.0], p16q=on}
      mask prompts: p3_4_5q "Power, Voltage and Frequency Ratings [MVA, kV, Hz]"; p7q "Primary and secondary voltage ratio [kV/kV]"; p8q "Resistance [p.u.]"; p9q "Reactance [p.u.]"; p11q "Fixed tap ratio [p.u./p.u.]"; p13_14_15q "Imax, Pmax and Smax  [p.u., p.u., p.u.]"; p16q "Connected"
      mask help: This block defines a transformer with constant tap ratio.
      mask init:
      | [x,y] = fm_draw('circle');
      | [x2,y2] = fm_draw('2');
      mask Callback p16q: fm_block
      mask Display:
      | plot(x,y,x+1.4,y,[-1 -1.3],[0 0],[2.4 2.7],[0 0])
      | color('green')
      | plot([-0.8 0.7],[-1.2 1.2],[0.5 0.7],[1.1 1.2],[0.7 0.7],[1.0 1.2])
      | plot(1.5+0.65*x2,0.65*y2)
  Transf2 : PMComponent  Tag=PSATblock  Description=Power Flow  PhysicalDomain=psatdomain  LeftPortType=p1  RightPortType=p1  LConnTagsString=__newl0  RConnTagsString=__newr0  mask(Line){p3_4_5q=[100  33  50], p7q=1, p8q=0.01, p9q=0.20, p13_14_15q=[0.0  0.0  0.0], p16q=on}
      mask prompts: p3_4_5q "Power, Voltage and Frequency Ratings [MVA, kV, Hz]"; p7q "Primary and secondary voltage ratio [kV/kV]"; p8q "Resistance [p.u.]"; p9q "Reactance [p.u.]"; p13_14_15q "Imax, Pmax and Smax [p.u., p.u., p.u.]"; p16q "Connected"
      mask help: This block defines a transformer.
      mask init:
      | [x,y] = fm_draw('circle');
      | [x1,y1] = fm_draw('1');
      | [x2,y2] = fm_draw('2');
      mask Callback p16q: fm_block
      mask Display:
      | plot(x,y,x+1.4,y,[-1 -1.3],[0 0],[2.4 2.7],[0 0])
      | color('green')
      | plot(-0.1+0.65*x1,0.65*y1)
      | plot(1.5+0.65*x2,0.65*y2)
  Transf5 : PMComponent  Tag=PSATblock  Description=Power Flow  PhysicalDomain=psatdomain  LeftPortType=p1  RightPortType=p1  LConnTagsString=__newl0  RConnTagsString=__newr0  mask(Line){p3_4_5q=[65  132  50], p7q=132/33, p8q=0, p9q=0.256, p11q=1.05, p13_14_15q=[0.0  0.0  0.0], p16q=on}
      mask prompts: p3_4_5q "Power, Voltage and Frequency Ratings [MVA, kV, Hz]"; p7q "Primary and secondary voltage ratio [kV/kV]"; p8q "Resistance [p.u.]"; p9q "Reactance [p.u.]"; p11q "Fixed tap ratio [p.u./p.u.]"; p13_14_15q "Imax, Pmax and Smax  [p.u., p.u., p.u.]"; p16q "Connected"
      mask help: This block defines a transformer with constant tap ratio.
      mask init:
      | [x,y] = fm_draw('circle');
      | [x2,y2] = fm_draw('2');
      mask Callback p16q: fm_block
      mask Display:
      | plot(x,y,x+1.4,y,[-1 -1.3],[0 0],[2.4 2.7],[0 0])
      | color('green')
      | plot([-0.8 0.7],[-1.2 1.2],[0.5 0.7],[1.1 1.2],[0.7 0.7],[1.0 1.2])
      | plot(1.5+0.65*x2,0.65*y2)
  Transf6 : PMComponent  Tag=PSATblock  Description=Power Flow  PhysicalDomain=psatdomain  LeftPortType=p1  RightPortType=p1  LConnTagsString=__newl0  RConnTagsString=__newr0  mask(Line){p3_4_5q=[65 33 50], p7q=33/132, p8q=0, p9q=0.369, p11q=1, p13_14_15q=[0.0  0.0  0.0], p16q=on}
      mask prompts: p3_4_5q "Power, Voltage and Frequency Ratings [MVA, kV, Hz]"; p7q "Primary and secondary voltage ratio [kV/kV]"; p8q "Resistance [p.u.]"; p9q "Reactance [p.u.]"; p11q "Fixed tap ratio [p.u./p.u.]"; p13_14_15q "Imax, Pmax and Smax  [p.u., p.u., p.u.]"; p16q "Connected"
      mask help: This block defines a transformer with constant tap ratio.
      mask init:
      | [x,y] = fm_draw('circle');
      | [x2,y2] = fm_draw('2');
      mask Callback p16q: fm_block
      mask Display:
      | plot(x,y,x+1.4,y,[-1 -1.3],[0 0],[2.4 2.7],[0 0])
      | color('green')
      | plot([-0.8 0.7],[-1.2 1.2],[0.5 0.7],[1.1 1.2],[0.7 0.7],[1.0 1.2])
      | plot(1.5+0.65*x2,0.65*y2)
  Wind : PMComponent  Tag=PSATblock  Description=Wind Turbines  PhysicalDomain=psatdomain  LeftPortType=p1  RightPortType=p1  RConnTagsString=__newr0  mask(Wind){out=1, p1q=measurements, p2q=15.00, p3q=1.225, p4q=4, p5q=0.1, p6_7q=[20  2], p8_9_10q=[5  15  1], p11_12_13q=[5  15  1], p14_15_16_17q=[50  0.01  0.2  50], p_18_19q=[10  1]}
      mask prompts: out "Number of output ports"; p1q "Wind model type"; p2q "Nominal wind speed [m/s]"; p3q "Air density rho [kg/m^3]"; p4q "Filter time constant tau [s]"; p5q "Sample time for wind measures [s]"; p6_7q "Weibull distribution constants  C and K"; p8_9_10q "Wind ramp constants Tsr, Ter and Awr [s s m/s]"; p11_12_13q "Wind gust constants Tsg, Teg and Awg [s s m/s]"; p14_15_16_17q "Wind turbolence constants h, z0, df and n [m - Hz int]"; p_18_19q "Mexican hat wavelet time center and shape factor"
      mask help: This block defines wind models for use with wind turbines.
      mask init:
      | fm_inout
      | [xa,ya] = fm_draw('arrow');
      mask TypeOptions p1q: measurements | weibull | composite | mexican_hat
      mask Display:
      | color('cyan')
      | plot(xa,ya,xa-0.2,ya-0.2,xa+0.2,ya+0.2,xa+0.4,ya+0.4,xa-0.4,ya-0.4)
  connections:
  Bus5/RConn3 -- PQ14/LConn1
  PQ16/LConn1 -- Bus7/LConn2
  Line39/LConn1 -- Bus5/RConn2
  Bus3/RConn2 -- PQ19/LConn1
  Line/LConn1 -- Bus01/RConn2
  Line7/RConn1 -- Bus01/RConn1
  Line7/LConn1 -- Bus2/RConn1
  PV/RConn1 -- Bus2/LConn2
  PQ/LConn1 -- Bus2/LConn1
  Line/RConn1 -- Bus3/LConn1
  PQ4/LConn1 -- Bus4/RConn2
  Bus2/RConn3 -- Line3/LConn1
  Line3/RConn1 -- Bus4/LConn2
  Bus3/RConn1 -- Line4/LConn1
  Line4/RConn1 -- Bus4/LConn1
  PV4/RConn1 -- Bus13/RConn1
  Bus14/RConn1 -- PQ22/LConn1
  Line26/LConn1 -- Bus12/RConn1
  Line26/RConn1 -- Bus14/LConn1
  Bus14/LConn2 -- Line27/LConn1
  Line27/RConn1 -- Bus15/LConn1
  Bus15/RConn1 -- PQ23/LConn1
  Bus15/LConn3 -- Line12/LConn1
  Line12/RConn1 -- Bus18/LConn1
  Line28/RConn1 -- Bus15/LConn2
  Bus12/RConn2 -- Line28/LConn1
  Bus16/RConn1 -- PQ24/LConn1
  Bus12/RConn3 -- Line14/LConn1
  Line14/RConn1 -- Bus16/LConn1
  Bus18/LConn2 -- Line18/LConn1
  Bus20/RConn1 -- Line29/LConn1
  Line29/RConn1 -- Bus19/LConn1
  Bus10/LConn2 -- Transf1/RConn1
  Bus17/LConn1 -- Line19/RConn1
  Line19/LConn1 -- Bus16/LConn2
  Line30/RConn1 -- Bus20/LConn1
  Line30/LConn1 -- Bus10/RConn1
  Line31/RConn1 -- Bus17/LConn2
  Bus10/RConn2 -- Line31/LConn1
  Line22/RConn1 -- Bus21/LConn1
  Bus10/RConn3 -- Line22/LConn1
  Bus22/LConn1 -- Line21/RConn1
  Line43/LConn1 -- Bus22/RConn1
  Line43/RConn1 -- Bus24/LConn2
  Bus18/RConn1 -- PQ25/LConn1
  PQ26/LConn1 -- Bus20/RConn2
  Bus21/RConn2 -- Line21/LConn1
  Line20/LConn1 -- Bus15/RConn2
  Line20/RConn1 -- Bus23/LConn1
  Bus23/RConn1 -- Line37/LConn1
  Line37/RConn1 -- Bus24/LConn1
  PQ17/LConn1 -- Bus17/RConn1
  PQ15/LConn1 -- Bus23/RConn2
  Bus30/RConn1 -- PQ11/LConn1
  Line44/RConn1 -- Bus27/RConn3
  PQ27/LConn1 -- Bus29/RConn1
  Line44/LConn1 -- Bus29/LConn2
  Line45/LConn1 -- Bus30/LConn2
  Line45/RConn1 -- Bus29/LConn1
  Bus30/LConn1 -- Line46/LConn1
  Line46/RConn1 -- Bus27/RConn2
  Line47/RConn1 -- Bus25/LConn2
  Line47/LConn1 -- Bus27/RConn1
  Bus24/RConn2 -- Line48/LConn1
  Line48/RConn1 -- Bus25/LConn1
  Bus27/LConn1 -- Transf6/LConn1
  Bus28/RConn1 -- Transf6/RConn1
  Line32/RConn1 -- Bus28/LConn2
  Bus26/RConn1 -- PQ18/LConn1
  Bus6/LConn5 -- Line25/LConn1
  Line25/RConn1 -- Bus28/LConn1
  Bus6/LConn4 -- Line34/LConn1
  Line34/RConn1 -- Bus8/RConn1
  PV3/RConn1 -- Bus11/RConn1
  Line38/LConn1 -- Bus7/RConn1
  Line38/RConn1 -- Bus6/LConn3
  Line17/LConn1 -- Bus2/RConn2
  Line17/RConn1 -- Bus6/LConn2
  Bus4/LConn3 -- Line16/LConn1
  Line16/RConn1 -- Bus6/LConn1
  Line39/RConn1 -- Bus7/LConn1
  Bus5/RConn1 -- Line15/RConn1
  Line15/LConn1 -- Bus2/LConn3
  PV1/RConn1 -- Bus5/LConn1
  PQ3/LConn1 -- Bus21/RConn1
  PQ5/LConn1 -- Bus10/RConn5
  Line2/RConn1 -- Bus22/LConn2
  Bus9/LConn1 -- Line6/RConn1
  Line18/RConn1 -- Bus19/RConn1
  PQ21/LConn1 -- Bus12/LConn3
  Bus12/LConn2 -- Transf5/RConn1
  Transf5/LConn1 -- Bus4/RConn1
  Bus10/RConn4 -- Line2/LConn1
  Bus25/RConn1 -- Line1/LConn1
  Line1/RConn1 -- Bus26/LConn1
  Transf1/LConn1 -- Bus6/RConn1
  Bus6/RConn2 -- Line6/LConn1
  Bus9/RConn1 -- Line9/LConn1
  Bus10/LConn1 -- Line9/RConn1
  Bus11/LConn1 -- Line8/RConn1
  Bus9/RConn2 -- Line8/LConn1
  Bus8/RConn2 -- Line32/LConn1
  PV2/RConn1 -- Bus8/LConn1
  Line5/LConn1 -- Bus13/LConn1
  Line5/RConn1 -- Bus12/LConn1
  PQ1/LConn1 -- Bus8/LConn2
  PQ6/LConn1 -- Bus19/LConn2
  Bus24/RConn1 -- PQ2/LConn1
  Slack/RConn1 -- Bus01/LConn1
  Shunt1/LConn1 -- Bus10/LConn3
  Shunt2/LConn1 -- Bus24/LConn3
  Dfig/LConn1 -- Wind/RConn1
  Dfig/RConn1 -- Bus1/RConn1
  Bus1/LConn2 -- Slack1/RConn1
  Bus1/LConn1 -- Transf2/LConn1
  Transf2/RConn1 -- Bus30/RConn2
